simulink model "model"  (R2014a)
(part 7 of 8)

  bus21 : powerlib/Measurements/Load Flow Bus  LConnTagsString=a  ID=bus21  Vbase=50000  Vref=1  Vangle=0  VLF=1  angleLF=0
      settings: AttributesFormatString=|
      | %<ID>
      | %<Vbase>V
      | %<VLF>pu
      | %<angleLF>deg.
      | %<Name>
  bus210 : powerlib/Measurements/Load Flow Bus  LConnTagsString=a  ID=bus210  Vbase=420000  Vref=1  Vangle=0  VLF=1  angleLF=0
      settings: AttributesFormatString=|
      | %<ID>
      | %<Vbase>V
      | %<VLF>pu
      | %<angleLF>deg.
      | %<Name>
  bus211 : powerlib/Measurements/Load Flow Bus  LConnTagsString=a  ID=bus211  Vbase=420000  Vref=1  Vangle=0  VLF=1  angleLF=0
      settings: AttributesFormatString=|
      | %<ID>
      | %<Vbase>V
      | %<VLF>pu
      | %<angleLF>deg.
      | %<Name>
  bus212 : powerlib/Measurements/Load Flow Bus  LConnTagsString=a  ID=bus212  Vbase=420000  Vref=1  Vangle=0  VLF=1  angleLF=0
      settings: AttributesFormatString=|
      | %<ID>
      | %<Vbase>V
      | %<VLF>pu
      | %<angleLF>deg.
      | %<Name>
  bus213 : powerlib/Measurements/Load Flow Bus  LConnTagsString=a  ID=bus213  Vbase=420000  Vref=1  Vangle=0  VLF=1  angleLF=0
      settings: AttributesFormatString=|
      | %<ID>
      | %<Vbase>V
      | %<VLF>pu
      | %<angleLF>deg.
      | %<Name>
  bus214 : powerlib/Measurements/Load Flow Bus  LConnTagsString=a  ID=bus214  Vbase=420000  Vref=1  Vangle=0  VLF=1  angleLF=0
      settings: AttributesFormatString=|
      | %<ID>
      | %<Vbase>V
      | %<VLF>pu
      | %<angleLF>deg.
      | %<Name>
  bus215 : powerlib/Measurements/Load Flow Bus  LConnTagsString=a  ID=bus215  Vbase=420000  Vref=1  Vangle=0  VLF=1  angleLF=0
      settings: AttributesFormatString=|
      | %<ID>
      | %<Vbase>V
      | %<VLF>pu
      | %<angleLF>deg.
      | %<Name>
  bus216 : powerlib/Measurements/Load Flow Bus  LConnTagsString=a  ID=bus216  Vbase=420000  Vref=1  Vangle=0  VLF=1  angleLF=0
      settings: AttributesFormatString=|
      | %<ID>
      | %<Vbase>V
      | %<VLF>pu
      | %<angleLF>deg.
      | %<Name>
  bus217 : powerlib/Measurements/Load Flow Bus  LConnTagsString=a  ID=bus217  Vbase=420000  Vref=1  Vangle=0  VLF=1  angleLF=0
      settings: AttributesFormatString=|
      | %<ID>
      | %<Vbase>V
      | %<VLF>pu
      | %<angleLF>deg.
      | %<Name>
  bus218 : powerlib/Measurements/Load Flow Bus  LConnTagsString=a  ID=bus218  Vbase=420000  Vref=1  Vangle=0  VLF=1  angleLF=0
      settings: AttributesFormatString=|
      | %<ID>
      | %<Vbase>V
      | %<VLF>pu
      | %<angleLF>deg.
      | %<Name>
  bus219 : powerlib/Measurements/Load Flow Bus  LConnTagsString=a  ID=bus219  Vbase=420000  Vref=1  Vangle=0  VLF=1  angleLF=0
      settings: AttributesFormatString=|
      | %<ID>
      | %<Vbase>V
      | %<VLF>pu
      | %<angleLF>deg.
      | %<Name>
  bus22 : powerlib/Measurements/Load Flow Bus  LConnTagsString=a  ID=bus22  Vbase=50000  Vref=1  Vangle=0  VLF=1  angleLF=0
      settings: AttributesFormatString=|
      | %<ID>
      | %<Vbase>V
      | %<VLF>pu
      | %<angleLF>deg.
      | %<Name>
  bus220 : powerlib/Measurements/Load Flow Bus  LConnTagsString=a  ID=bus220  Vbase=420000  Vref=1  Vangle=0  VLF=1  angleLF=0
      settings: AttributesFormatString=|
      | %<ID>
      | %<Vbase>V
      | %<VLF>pu
      | %<angleLF>deg.
      | %<Name>
  bus221 : powerlib/Measurements/Load Flow Bus  LConnTagsString=a  ID=bus221  Vbase=420000  Vref=1  Vangle=0  VLF=1  angleLF=0
      settings: AttributesFormatString=|
      | %<ID>
      | %<Vbase>V
      | %<VLF>pu
      | %<angleLF>deg.
      | %<Name>
  bus222 : powerlib/Measurements/Load Flow Bus  LConnTagsString=a  ID=bus222  Vbase=420000  Vref=1  Vangle=0  VLF=1  angleLF=0
      settings: AttributesFormatString=|
      | %<ID>
      | %<Vbase>V
      | %<VLF>pu
      | %<angleLF>deg.
      | %<Name>
  bus223 : powerlib/Measurements/Load Flow Bus  LConnTagsString=a  ID=bus223  Vbase=420000  Vref=1  Vangle=0  VLF=1  angleLF=0
      settings: AttributesFormatString=|
      | %<ID>
      | %<Vbase>V
      | %<VLF>pu
      | %<angleLF>deg.
      | %<Name>
  bus224 : powerlib/Measurements/Load Flow Bus  LConnTagsString=a  ID=bus224  Vbase=420000  Vref=1  Vangle=0  VLF=1  angleLF=0
      settings: AttributesFormatString=|
      | %<ID>
      | %<Vbase>V
      | %<VLF>pu
      | %<angleLF>deg.
      | %<Name>
  bus225 : powerlib/Measurements/Load Flow Bus  LConnTagsString=a  ID=bus225  Vbase=420000  Vref=1  Vangle=0  VLF=1  angleLF=0
      settings: AttributesFormatString=|
      | %<ID>
      | %<Vbase>V
      | %<VLF>pu
      | %<angleLF>deg.
      | %<Name>
  bus226 : powerlib/Measurements/Load Flow Bus  LConnTagsString=a  ID=bus226  Vbase=420000  Vref=1  Vangle=0  VLF=1  angleLF=0
      settings: AttributesFormatString=|
      | %<ID>
      | %<Vbase>V
      | %<VLF>pu
      | %<angleLF>deg.
      | %<Name>
  bus227 : powerlib/Measurements/Load Flow Bus  LConnTagsString=a  ID=bus227  Vbase=420000  Vref=1  Vangle=0  VLF=1  angleLF=0
      settings: AttributesFormatString=|
      | %<ID>
      | %<Vbase>V
      | %<VLF>pu
      | %<angleLF>deg.
      | %<Name>
  bus228 : powerlib/Measurements/Load Flow Bus  LConnTagsString=a  ID=bus228  Vbase=50000  Vref=1  Vangle=0  VLF=1  angleLF=0
      settings: AttributesFormatString=|
      | %<ID>
      | %<Vbase>V
      | %<VLF>pu
      | %<angleLF>deg.
      | %<Name>
  bus229 : powerlib/Measurements/Load Flow Bus  LConnTagsString=a  ID=bus229  Vbase=50000  Vref=1  Vangle=0  VLF=1  angleLF=0
      settings: AttributesFormatString=|
      | %<ID>
      | %<Vbase>V
      | %<VLF>pu
      | %<angleLF>deg.
      | %<Name>
  bus23 : powerlib/Measurements/Load Flow Bus  LConnTagsString=a  ID=bus23  Vbase=50000  Vref=1  Vangle=0  VLF=1  angleLF=0
      settings: AttributesFormatString=|
      | %<ID>
      | %<Vbase>V
      | %<VLF>pu
      | %<angleLF>deg.
      | %<Name>
  bus230 : powerlib/Measurements/Load Flow Bus  LConnTagsString=a  ID=bus230  Vbase=50000  Vref=1  Vangle=0  VLF=1  angleLF=0
      settings: AttributesFormatString=|
      | %<ID>
      | %<Vbase>V
      | %<VLF>pu
      | %<angleLF>deg.
      | %<Name>
  bus231 : powerlib/Measurements/Load Flow Bus  LConnTagsString=a  ID=bus231  Vbase=50000  Vref=1  Vangle=0  VLF=1  angleLF=0
      settings: AttributesFormatString=|
      | %<ID>
      | %<Vbase>V
      | %<VLF>pu
      | %<angleLF>deg.
      | %<Name>
  bus232 : powerlib/Measurements/Load Flow Bus  LConnTagsString=a  ID=bus232  Vbase=50000  Vref=1  Vangle=0  VLF=1  angleLF=0
      settings: AttributesFormatString=|
      | %<ID>
      | %<Vbase>V
      | %<VLF>pu
      | %<angleLF>deg.
      | %<Name>
  bus233 : powerlib/Measurements/Load Flow Bus  LConnTagsString=a  ID=bus233  Vbase=50000  Vref=1  Vangle=0  VLF=1  angleLF=0
      settings: AttributesFormatString=|
      | %<ID>
      | %<Vbase>V
      | %<VLF>pu
      | %<angleLF>deg.
      | %<Name>
  bus234 : powerlib/Measurements/Load Flow Bus  LConnTagsString=a  ID=bus234  Vbase=50000  Vref=1  Vangle=0  VLF=1  angleLF=0
      settings: AttributesFormatString=|
      | %<ID>
      | %<Vbase>V
      | %<VLF>pu
      | %<angleLF>deg.
      | %<Name>
  bus235 : powerlib/Measurements/Load Flow Bus  LConnTagsString=a  ID=bus235  Vbase=50000  Vref=1  Vangle=0  VLF=1  angleLF=0
      settings: AttributesFormatString=|
      | %<ID>
      | %<Vbase>V
      | %<VLF>pu
      | %<angleLF>deg.
      | %<Name>
  bus236 : powerlib/Measurements/Load Flow Bus  LConnTagsString=a  ID=bus236  Vbase=50000  Vref=1  Vangle=0  VLF=1  angleLF=0
      settings: AttributesFormatString=|
      | %<ID>
      | %<Vbase>V
      | %<VLF>pu
      | %<angleLF>deg.
      | %<Name>
  bus237 : powerlib/Measurements/Load Flow Bus  LConnTagsString=a  ID=bus237  Vbase=50000  Vref=1  Vangle=0  VLF=1  angleLF=0
      settings: AttributesFormatString=|
      | %<ID>
      | %<Vbase>V
      | %<VLF>pu
      | %<angleLF>deg.
      | %<Name>
  bus238 : powerlib/Measurements/Load Flow Bus  LConnTagsString=a  ID=bus238  Vbase=50000  Vref=1  Vangle=0  VLF=1  angleLF=0
      settings: AttributesFormatString=|
      | %<ID>
      | %<Vbase>V
      | %<VLF>pu
      | %<angleLF>deg.
      | %<Name>
  bus239 : powerlib/Measurements/Load Flow Bus  LConnTagsString=a  ID=bus239  Vbase=50000  Vref=1  Vangle=0  VLF=1  angleLF=0
      settings: AttributesFormatString=|
      | %<ID>
      | %<Vbase>V
      | %<VLF>pu
      | %<angleLF>deg.
      | %<Name>
  bus24 : powerlib/Measurements/Load Flow Bus  LConnTagsString=a  ID=bus24  Vbase=50000  Vref=1  Vangle=0  VLF=1  angleLF=0
      settings: AttributesFormatString=|
      | %<ID>
      | %<Vbase>V
      | %<VLF>pu
      | %<angleLF>deg.
      | %<Name>
  bus240 : powerlib/Measurements/Load Flow Bus  LConnTagsString=a  ID=bus240  Vbase=50000  Vref=1  Vangle=0  VLF=1  angleLF=0
      settings: AttributesFormatString=|
      | %<ID>
      | %<Vbase>V
      | %<VLF>pu
      | %<angleLF>deg.
      | %<Name>
  bus241 : powerlib/Measurements/Load Flow Bus  LConnTagsString=a  ID=bus241  Vbase=50000  Vref=1  Vangle=0  VLF=1  angleLF=0
      settings: AttributesFormatString=|
      | %<ID>
      | %<Vbase>V
      | %<VLF>pu
      | %<angleLF>deg.
      | %<Name>
  bus242 : powerlib/Measurements/Load Flow Bus  LConnTagsString=a  ID=bus242  Vbase=50000  Vref=1  Vangle=0  VLF=1  angleLF=0
      settings: AttributesFormatString=|
      | %<ID>
      | %<Vbase>V
      | %<VLF>pu
      | %<angleLF>deg.
      | %<Name>
  bus243 : powerlib/Measurements/Load Flow Bus  LConnTagsString=a  ID=bus243  Vbase=50000  Vref=1  Vangle=0  VLF=1  angleLF=0
      settings: AttributesFormatString=|
      | %<ID>
      | %<Vbase>V
      | %<VLF>pu
      | %<angleLF>deg.
      | %<Name>
  bus244 : powerlib/Measurements/Load Flow Bus  LConnTagsString=a  ID=bus244  Vbase=50000  Vref=1  Vangle=0  VLF=1  angleLF=0
      settings: AttributesFormatString=|
      | %<ID>
      | %<Vbase>V
      | %<VLF>pu
      | %<angleLF>deg.
      | %<Name>
  bus245 : powerlib/Measurements/Load Flow Bus  LConnTagsString=a  ID=bus245  Vbase=50000  Vref=1  Vangle=0  VLF=1  angleLF=0
      settings: AttributesFormatString=|
      | %<ID>
      | %<Vbase>V
      | %<VLF>pu
      | %<angleLF>deg.
      | %<Name>
  bus246 : powerlib/Measurements/Load Flow Bus  LConnTagsString=a  ID=bus246  Vbase=50000  Vref=1  Vangle=0  VLF=1  angleLF=0
      settings: AttributesFormatString=|
      | %<ID>
      | %<Vbase>V
      | %<VLF>pu
      | %<angleLF>deg.
      | %<Name>
  bus247 : powerlib/Measurements/Load Flow Bus  LConnTagsString=a  ID=bus247  Vbase=50000  Vref=1  Vangle=0  VLF=1  angleLF=0
      settings: AttributesFormatString=|
      | %<ID>
      | %<Vbase>V
      | %<VLF>pu
      | %<angleLF>deg.
      | %<Name>
  bus248 : powerlib/Measurements/Load Flow Bus  LConnTagsString=a  ID=bus248  Vbase=50000  Vref=1  Vangle=0  VLF=1  angleLF=0
      settings: AttributesFormatString=|
      | %<ID>
      | %<Vbase>V
      | %<VLF>pu
      | %<angleLF>deg.
      | %<Name>
  bus249 : powerlib/Measurements/Load Flow Bus  LConnTagsString=a  ID=bus249  Vbase=50000  Vref=1  Vangle=0  VLF=1  angleLF=0
      settings: AttributesFormatString=|
      | %<ID>
      | %<Vbase>V
      | %<VLF>pu
      | %<angleLF>deg.
      | %<Name>
  bus25 : powerlib/Measurements/Load Flow Bus  LConnTagsString=a  ID=bus25  Vbase=50000  Vref=1  Vangle=0  VLF=1  angleLF=0
      settings: AttributesFormatString=|
      | %<ID>
      | %<Vbase>V
      | %<VLF>pu
      | %<angleLF>deg.
      | %<Name>
  bus250 : powerlib/Measurements/Load Flow Bus  LConnTagsString=a  ID=bus250  Vbase=50000  Vref=1  Vangle=0  VLF=1  angleLF=0
      settings: AttributesFormatString=|
      | %<ID>
      | %<Vbase>V
      | %<VLF>pu
      | %<angleLF>deg.
      | %<Name>
  bus251 : powerlib/Measurements/Load Flow Bus  LConnTagsString=a  ID=bus251  Vbase=50000  Vref=1  Vangle=0  VLF=1  angleLF=0
      settings: AttributesFormatString=|
      | %<ID>
      | %<Vbase>V
      | %<VLF>pu
      | %<angleLF>deg.
      | %<Name>
  bus252 : powerlib/Measurements/Load Flow Bus  LConnTagsString=a  ID=bus252  Vbase=50000  Vref=1  Vangle=0  VLF=1  angleLF=0
      settings: AttributesFormatString=|
      | %<ID>
      | %<Vbase>V
      | %<VLF>pu
      | %<angleLF>deg.
      | %<Name>
  bus253 : powerlib/Measurements/Load Flow Bus  LConnTagsString=a  ID=bus253  Vbase=50000  Vref=1  Vangle=0  VLF=1  angleLF=0
      settings: AttributesFormatString=|
      | %<ID>
      | %<Vbase>V
      | %<VLF>pu
      | %<angleLF>deg.
      | %<Name>
  bus254 : powerlib/Measurements/Load Flow Bus  LConnTagsString=a  ID=bus254  Vbase=50000  Vref=1  Vangle=0  VLF=1  angleLF=0
      settings: AttributesFormatString=|
      | %<ID>
      | %<Vbase>V
      | %<VLF>pu
      | %<angleLF>deg.
      | %<Name>
  bus255 : powerlib/Measurements/Load Flow Bus  LConnTagsString=a  ID=bus255  Vbase=50000  Vref=1  Vangle=0  VLF=1  angleLF=0
      settings: AttributesFormatString=|
      | %<ID>
      | %<Vbase>V
      | %<VLF>pu
      | %<angleLF>deg.
      | %<Name>
  bus256 : powerlib/Measurements/Load Flow Bus  LConnTagsString=a  ID=bus256  Vbase=66000  Vref=1  Vangle=0  VLF=1  angleLF=0
      settings: AttributesFormatString=|
      | %<ID>
      | %<Vbase>V
      | %<VLF>pu
      | %<angleLF>deg.
      | %<Name>
  bus257 : powerlib/Measurements/Load Flow Bus  LConnTagsString=a  ID=bus257  Vbase=66000  Vref=1  Vangle=0  VLF=1  angleLF=0
      settings: AttributesFormatString=|
      | %<ID>
      | %<Vbase>V
      | %<VLF>pu
      | %<angleLF>deg.
      | %<Name>
  bus258 : powerlib/Measurements/Load Flow Bus  LConnTagsString=a  ID=bus258  Vbase=66000  Vref=1  Vangle=0  VLF=1  angleLF=0
      settings: AttributesFormatString=|
      | %<ID>
      | %<Vbase>V
      | %<VLF>pu
      | %<angleLF>deg.
      | %<Name>
  bus259 : powerlib/Measurements/Load Flow Bus  LConnTagsString=a  ID=bus259  Vbase=66000  Vref=1  Vangle=0  VLF=1  angleLF=0
      settings: AttributesFormatString=|
      | %<ID>
      | %<Vbase>V
      | %<VLF>pu
      | %<angleLF>deg.
      | %<Name>
  bus26 : powerlib/Measurements/Load Flow Bus  LConnTagsString=a  ID=bus26  Vbase=50000  Vref=1  Vangle=0  VLF=1  angleLF=0
      settings: AttributesFormatString=|
      | %<ID>
      | %<Vbase>V
      | %<VLF>pu
      | %<angleLF>deg.
      | %<Name>
  bus260 : powerlib/Measurements/Load Flow Bus  LConnTagsString=a  ID=bus260  Vbase=66000  Vref=1  Vangle=0  VLF=1  angleLF=0
      settings: AttributesFormatString=|
      | %<ID>
      | %<Vbase>V
      | %<VLF>pu
      | %<angleLF>deg.
      | %<Name>
  bus261 : powerlib/Measurements/Load Flow Bus  LConnTagsString=a  ID=bus261  Vbase=66000  Vref=1  Vangle=0  VLF=1  angleLF=0
      settings: AttributesFormatString=|
      | %<ID>
      | %<Vbase>V
      | %<VLF>pu
      | %<angleLF>deg.
      | %<Name>
  bus262 : powerlib/Measurements/Load Flow Bus  LConnTagsString=a  ID=bus262  Vbase=66000  Vref=1  Vangle=0  VLF=1  angleLF=0
      settings: AttributesFormatString=|
      | %<ID>
      | %<Vbase>V
      | %<VLF>pu
      | %<angleLF>deg.
      | %<Name>
  bus263 : powerlib/Measurements/Load Flow Bus  LConnTagsString=a  ID=bus263  Vbase=66000  Vref=1  Vangle=0  VLF=1  angleLF=0
      settings: AttributesFormatString=|
      | %<ID>
      | %<Vbase>V
      | %<VLF>pu
      | %<angleLF>deg.
      | %<Name>
  bus264 : powerlib/Measurements/Load Flow Bus  LConnTagsString=a  ID=bus264  Vbase=66000  Vref=1  Vangle=0  VLF=1  angleLF=0
      settings: AttributesFormatString=|
      | %<ID>
      | %<Vbase>V
      | %<VLF>pu
      | %<angleLF>deg.
      | %<Name>
  bus265 : powerlib/Measurements/Load Flow Bus  LConnTagsString=a  ID=bus265  Vbase=66000  Vref=1  Vangle=0  VLF=1  angleLF=0
      settings: AttributesFormatString=|
      | %<ID>
      | %<Vbase>V
      | %<VLF>pu
      | %<angleLF>deg.
      | %<Name>
  bus266 : powerlib/Measurements/Load Flow Bus  LConnTagsString=a  ID=bus266  Vbase=66000  Vref=1  Vangle=0  VLF=1  angleLF=0
      settings: AttributesFormatString=|
      | %<ID>
      | %<Vbase>V
      | %<VLF>pu
      | %<angleLF>deg.
      | %<Name>
  bus267 : powerlib/Measurements/Load Flow Bus  LConnTagsString=a  ID=bus267  Vbase=66000  Vref=1  Vangle=0  VLF=1  angleLF=0
      settings: AttributesFormatString=|
      | %<ID>
      | %<Vbase>V
      | %<VLF>pu
      | %<angleLF>deg.
      | %<Name>
  bus268 : powerlib/Measurements/Load Flow Bus  LConnTagsString=a  ID=bus268  Vbase=66000  Vref=1  Vangle=0  VLF=1  angleLF=0
      settings: AttributesFormatString=|
      | %<ID>
      | %<Vbase>V
      | %<VLF>pu
      | %<angleLF>deg.
      | %<Name>
  bus269 : powerlib/Measurements/Load Flow Bus  LConnTagsString=a  ID=bus269  Vbase=132000  Vref=1  Vangle=0  VLF=1  angleLF=0
      settings: AttributesFormatString=|
      | %<ID>
      | %<Vbase>V
      | %<VLF>pu
      | %<angleLF>deg.
      | %<Name>
  bus27 : powerlib/Measurements/Load Flow Bus  LConnTagsString=a  ID=bus27  Vbase=50000  Vref=1  Vangle=0  VLF=1  angleLF=0
      settings: AttributesFormatString=|
      | %<ID>
      | %<Vbase>V
      | %<VLF>pu
      | %<angleLF>deg.
      | %<Name>
  bus270 : powerlib/Measurements/Load Flow Bus  LConnTagsString=a  ID=bus270  Vbase=132000  Vref=1  Vangle=0  VLF=1  angleLF=0
      settings: AttributesFormatString=|
      | %<ID>
      | %<Vbase>V
      | %<VLF>pu
      | %<angleLF>deg.
      | %<Name>
  bus271 : powerlib/Measurements/Load Flow Bus  LConnTagsString=a  ID=bus271  Vbase=132000  Vref=1  Vangle=0  VLF=1  angleLF=0
      settings: AttributesFormatString=|
      | %<ID>
      | %<Vbase>V
      | %<VLF>pu
      | %<angleLF>deg.
      | %<Name>
  bus272 : powerlib/Measurements/Load Flow Bus  LConnTagsString=a  ID=bus272  Vbase=132000  Vref=1  Vangle=0  VLF=1  angleLF=0
      settings: AttributesFormatString=|
      | %<ID>
      | %<Vbase>V
      | %<VLF>pu
      | %<angleLF>deg.
      | %<Name>
  bus273 : powerlib/Measurements/Load Flow Bus  LConnTagsString=a  ID=bus273  Vbase=132000  Vref=1  Vangle=0  VLF=1  angleLF=0
      settings: AttributesFormatString=|
      | %<ID>
      | %<Vbase>V
      | %<VLF>pu
      | %<angleLF>deg.
      | %<Name>
  bus274 : powerlib/Measurements/Load Flow Bus  LConnTagsString=a  ID=bus274  Vbase=132000  Vref=1  Vangle=0  VLF=1  angleLF=0
      settings: AttributesFormatString=|
      | %<ID>
      | %<Vbase>V
      | %<VLF>pu
      | %<angleLF>deg.
      | %<Name>
  bus275 : powerlib/Measurements/Load Flow Bus  LConnTagsString=a  ID=bus275  Vbase=132000  Vref=1  Vangle=0  VLF=1  angleLF=0
      settings: AttributesFormatString=|
      | %<ID>
      | %<Vbase>V
      | %<VLF>pu
      | %<angleLF>deg.
      | %<Name>
  bus276 : powerlib/Measurements/Load Flow Bus  LConnTagsString=a  ID=bus276  Vbase=132000  Vref=1  Vangle=0  VLF=1  angleLF=0
      settings: AttributesFormatString=|
      | %<ID>
      | %<Vbase>V
      | %<VLF>pu
      | %<angleLF>deg.
      | %<Name>
  bus277 : powerlib/Measurements/Load Flow Bus  LConnTagsString=a  ID=bus277  Vbase=132000  Vref=1  Vangle=0  VLF=1  angleLF=0
      settings: AttributesFormatString=|
      | %<ID>
      | %<Vbase>V
      | %<VLF>pu
      | %<angleLF>deg.
      | %<Name>
  bus278 : powerlib/Measurements/Load Flow Bus  LConnTagsString=a  ID=bus278  Vbase=132000  Vref=1  Vangle=0  VLF=1  angleLF=0
      settings: AttributesFormatString=|
      | %<ID>
      | %<Vbase>V
      | %<VLF>pu
      | %<angleLF>deg.
      | %<Name>
  bus279 : powerlib/Measurements/Load Flow Bus  LConnTagsString=a  ID=bus279  Vbase=132000  Vref=1  Vangle=0  VLF=1  angleLF=0
      settings: AttributesFormatString=|
      | %<ID>
      | %<Vbase>V
      | %<VLF>pu
      | %<angleLF>deg.
      | %<Name>
  bus28 : powerlib/Measurements/Load Flow Bus  LConnTagsString=a  ID=bus28  Vbase=50000  Vref=1  Vangle=0  VLF=1  angleLF=0
      settings: AttributesFormatString=|
      | %<ID>
      | %<Vbase>V
      | %<VLF>pu
      | %<angleLF>deg.
      | %<Name>
  bus280 : powerlib/Measurements/Load Flow Bus  LConnTagsString=a  ID=bus280  Vbase=132000  Vref=1  Vangle=0  VLF=1  angleLF=0
      settings: AttributesFormatString=|
      | %<ID>
      | %<Vbase>V
      | %<VLF>pu
      | %<angleLF>deg.
      | %<Name>
  bus281 : powerlib/Measurements/Load Flow Bus  LConnTagsString=a  ID=bus281  Vbase=132000  Vref=1  Vangle=0  VLF=1  angleLF=0
      settings: AttributesFormatString=|
      | %<ID>
      | %<Vbase>V
      | %<VLF>pu
      | %<angleLF>deg.
      | %<Name>
  bus282 : powerlib/Measurements/Load Flow Bus  LConnTagsString=a  ID=bus282  Vbase=132000  Vref=1  Vangle=0  VLF=1  angleLF=0
      settings: AttributesFormatString=|
      | %<ID>
      | %<Vbase>V
      | %<VLF>pu
      | %<angleLF>deg.
      | %<Name>
  bus283 : powerlib/Measurements/Load Flow Bus  LConnTagsString=a  ID=bus283  Vbase=132000  Vref=1  Vangle=0  VLF=1  angleLF=0
      settings: AttributesFormatString=|
      | %<ID>
      | %<Vbase>V
      | %<VLF>pu
      | %<angleLF>deg.
      | %<Name>
  bus284 : powerlib/Measurements/Load Flow Bus  LConnTagsString=a  ID=bus284  Vbase=132000  Vref=1  Vangle=0  VLF=1  angleLF=0
      settings: AttributesFormatString=|
      | %<ID>
      | %<Vbase>V
      | %<VLF>pu
      | %<angleLF>deg.
      | %<Name>
  bus285 : powerlib/Measurements/Load Flow Bus  LConnTagsString=a  ID=bus285  Vbase=132000  Vref=1  Vangle=0  VLF=1  angleLF=0
      settings: AttributesFormatString=|
      | %<ID>
      | %<Vbase>V
      | %<VLF>pu
      | %<angleLF>deg.
      | %<Name>
  bus286 : powerlib/Measurements/Load Flow Bus  LConnTagsString=a  ID=bus286  Vbase=132000  Vref=1  Vangle=0  VLF=1  angleLF=0
      settings: AttributesFormatString=|
      | %<ID>
      | %<Vbase>V
      | %<VLF>pu
      | %<angleLF>deg.
      | %<Name>
  bus287 : powerlib/Measurements/Load Flow Bus  LConnTagsString=a  ID=bus287  Vbase=132000  Vref=1  Vangle=0  VLF=1  angleLF=0
      settings: AttributesFormatString=|
      | %<ID>
      | %<Vbase>V
      | %<VLF>pu
      | %<angleLF>deg.
      | %<Name>
  bus288 : powerlib/Measurements/Load Flow Bus  LConnTagsString=a  ID=bus288  Vbase=132000  Vref=1  Vangle=0  VLF=1  angleLF=0
      settings: AttributesFormatString=|
      | %<ID>
      | %<Vbase>V
      | %<VLF>pu
      | %<angleLF>deg.
      | %<Name>
  bus289 : powerlib/Measurements/Load Flow Bus  LConnTagsString=a  ID=bus289  Vbase=132000  Vref=1  Vangle=0  VLF=1  angleLF=0
      settings: AttributesFormatString=|
      | %<ID>
      | %<Vbase>V
      | %<VLF>pu
      | %<angleLF>deg.
      | %<Name>
  bus29 : powerlib/Measurements/Load Flow Bus  LConnTagsString=a  ID=bus29  Vbase=50000  Vref=1  Vangle=0  VLF=1  angleLF=0
      settings: AttributesFormatString=|
      | %<ID>
      | %<Vbase>V
      | %<VLF>pu
      | %<angleLF>deg.
      | %<Name>
  bus290 : powerlib/Measurements/Load Flow Bus  LConnTagsString=a  ID=bus290  Vbase=132000  Vref=1  Vangle=0  VLF=1  angleLF=0
      settings: AttributesFormatString=|
      | %<ID>
      | %<Vbase>V
      | %<VLF>pu
      | %<angleLF>deg.
      | %<Name>
  bus291 : powerlib/Measurements/Load Flow Bus  LConnTagsString=a  ID=bus291  Vbase=132000  Vref=1  Vangle=0  VLF=1  angleLF=0
      settings: AttributesFormatString=|
      | %<ID>
      | %<Vbase>V
      | %<VLF>pu
      | %<angleLF>deg.
      | %<Name>
  bus292 : powerlib/Measurements/Load Flow Bus  LConnTagsString=a  ID=bus292  Vbase=132000  Vref=1  Vangle=0  VLF=1  angleLF=0
      settings: AttributesFormatString=|
      | %<ID>
      | %<Vbase>V
      | %<VLF>pu
      | %<angleLF>deg.
      | %<Name>
  bus293 : powerlib/Measurements/Load Flow Bus  LConnTagsString=a  ID=bus293  Vbase=132000  Vref=1  Vangle=0  VLF=1  angleLF=0
      settings: AttributesFormatString=|
      | %<ID>
      | %<Vbase>V
      | %<VLF>pu
      | %<angleLF>deg.
      | %<Name>
  bus294 : powerlib/Measurements/Load Flow Bus  LConnTagsString=a  ID=bus294  Vbase=132000  Vref=1  Vangle=0  VLF=1  angleLF=0
      settings: AttributesFormatString=|
      | %<ID>
      | %<Vbase>V
      | %<VLF>pu
      | %<angleLF>deg.
      | %<Name>
  bus295 : powerlib/Measurements/Load Flow Bus  LConnTagsString=a  ID=bus295  Vbase=132000  Vref=1  Vangle=0  VLF=1  angleLF=0
      settings: AttributesFormatString=|
      | %<ID>
      | %<Vbase>V
      | %<VLF>pu
      | %<angleLF>deg.
      | %<Name>
  bus296 : powerlib/Measurements/Load Flow Bus  LConnTagsString=a  ID=bus296  Vbase=132000  Vref=1  Vangle=0  VLF=1  angleLF=0
      settings: AttributesFormatString=|
      | %<ID>
      | %<Vbase>V
      | %<VLF>pu
      | %<angleLF>deg.
      | %<Name>
  bus297 : powerlib/Measurements/Load Flow Bus  LConnTagsString=a  ID=bus297  Vbase=132000  Vref=1  Vangle=0  VLF=1  angleLF=0
      settings: AttributesFormatString=|
      | %<ID>
      | %<Vbase>V
      | %<VLF>pu
      | %<angleLF>deg.
      | %<Name>
  bus298 : powerlib/Measurements/Load Flow Bus  LConnTagsString=a  ID=bus298  Vbase=132000  Vref=1  Vangle=0  VLF=1  angleLF=0
      settings: AttributesFormatString=|
      | %<ID>
      | %<Vbase>V
      | %<VLF>pu
      | %<angleLF>deg.
      | %<Name>
  bus299 : powerlib/Measurements/Load Flow Bus  LConnTagsString=a  ID=bus299  Vbase=132000  Vref=1  Vangle=0  VLF=1  angleLF=0
      settings: AttributesFormatString=|
      | %<ID>
      | %<Vbase>V
      | %<VLF>pu
      | %<angleLF>deg.
      | %<Name>
  bus3 : powerlib/Measurements/Load Flow Bus  LConnTagsString=a  ID=bus3  Vbase=50000  Vref=1  Vangle=0  VLF=1  angleLF=0
      settings: AttributesFormatString=|
      | %<ID>
      | %<Vbase>V
      | %<VLF>pu
      | %<angleLF>deg.
      | %<Name>
  bus30 : powerlib/Measurements/Load Flow Bus  LConnTagsString=a  ID=bus30  Vbase=50000  Vref=1  Vangle=0  VLF=1  angleLF=0
      settings: AttributesFormatString=|
      | %<ID>
      | %<Vbase>V
      | %<VLF>pu
      | %<angleLF>deg.
      | %<Name>
  bus300 : powerlib/Measurements/Load Flow Bus  LConnTagsString=a  ID=bus300  Vbase=132000  Vref=1  Vangle=0  VLF=1  angleLF=0
      settings: AttributesFormatString=|
      | %<ID>
      | %<Vbase>V
      | %<VLF>pu
      | %<angleLF>deg.
      | %<Name>
  bus301 : powerlib/Measurements/Load Flow Bus  LConnTagsString=a  ID=bus301  Vbase=132000  Vref=1  Vangle=0  VLF=1  angleLF=0
      settings: AttributesFormatString=|
      | %<ID>
      | %<Vbase>V
      | %<VLF>pu
      | %<angleLF>deg.
      | %<Name>
  bus302 : powerlib/Measurements/Load Flow Bus  LConnTagsString=a  ID=bus302  Vbase=132000  Vref=1  Vangle=0  VLF=1  angleLF=0
      settings: AttributesFormatString=|
      | %<ID>
      | %<Vbase>V
      | %<VLF>pu
      | %<angleLF>deg.
      | %<Name>
  bus303 : powerlib/Measurements/Load Flow Bus  LConnTagsString=a  ID=bus303  Vbase=132000  Vref=1  Vangle=0  VLF=1  angleLF=0
      settings: AttributesFormatString=|
      | %<ID>
      | %<Vbase>V
      | %<VLF>pu
      | %<angleLF>deg.
      | %<Name>
  bus304 : powerlib/Measurements/Load Flow Bus  LConnTagsString=a  ID=bus304  Vbase=132000  Vref=1  Vangle=0  VLF=1  angleLF=0
      settings: AttributesFormatString=|
      | %<ID>
      | %<Vbase>V
      | %<VLF>pu
      | %<angleLF>deg.
      | %<Name>
  bus305 : powerlib/Measurements/Load Flow Bus  LConnTagsString=a  ID=bus305  Vbase=132000  Vref=1  Vangle=0  VLF=1  angleLF=0
      settings: AttributesFormatString=|
      | %<ID>
      | %<Vbase>V
      | %<VLF>pu
      | %<angleLF>deg.
      | %<Name>
  bus306 : powerlib/Measurements/Load Flow Bus  LConnTagsString=a  ID=bus306  Vbase=132000  Vref=1  Vangle=0  VLF=1  angleLF=0
      settings: AttributesFormatString=|
      | %<ID>
      | %<Vbase>V
      | %<VLF>pu
      | %<angleLF>deg.
      | %<Name>
  bus307 : powerlib/Measurements/Load Flow Bus  LConnTagsString=a  ID=bus307  Vbase=132000  Vref=1  Vangle=0  VLF=1  angleLF=0
      settings: AttributesFormatString=|
      | %<ID>
      | %<Vbase>V
      | %<VLF>pu
      | %<angleLF>deg.
      | %<Name>
  bus308 : powerlib/Measurements/Load Flow Bus  LConnTagsString=a  ID=bus308  Vbase=132000  Vref=1  Vangle=0  VLF=1  angleLF=0
      settings: AttributesFormatString=|
      | %<ID>
      | %<Vbase>V
      | %<VLF>pu
      | %<angleLF>deg.
      | %<Name>
  bus309 : powerlib/Measurements/Load Flow Bus  LConnTagsString=a  ID=bus309  Vbase=132000  Vref=1  Vangle=0  VLF=1  angleLF=0
      settings: AttributesFormatString=|
      | %<ID>
      | %<Vbase>V
      | %<VLF>pu
      | %<angleLF>deg.
      | %<Name>
  bus31 : powerlib/Measurements/Load Flow Bus  LConnTagsString=a  ID=bus31  Vbase=50000  Vref=1  Vangle=0  VLF=1  angleLF=0
      settings: AttributesFormatString=|
      | %<ID>
      | %<Vbase>V
      | %<VLF>pu
      | %<angleLF>deg.
      | %<Name>
  bus310 : powerlib/Measurements/Load Flow Bus  LConnTagsString=a  ID=bus310  Vbase=132000  Vref=1  Vangle=0  VLF=1  angleLF=0
      settings: AttributesFormatString=|
      | %<ID>
      | %<Vbase>V
      | %<VLF>pu
      | %<angleLF>deg.
      | %<Name>
  bus311 : powerlib/Measurements/Load Flow Bus  LConnTagsString=a  ID=bus311  Vbase=132000  Vref=1  Vangle=0  VLF=1  angleLF=0
      settings: AttributesFormatString=|
      | %<ID>
      | %<Vbase>V
      | %<VLF>pu
      | %<angleLF>deg.
      | %<Name>
  bus312 : powerlib/Measurements/Load Flow Bus  LConnTagsString=a  ID=bus312  Vbase=132000  Vref=1  Vangle=0  VLF=1  angleLF=0
      settings: AttributesFormatString=|
      | %<ID>
      | %<Vbase>V
      | %<VLF>pu
      | %<angleLF>deg.
      | %<Name>
  bus313 : powerlib/Measurements/Load Flow Bus  LConnTagsString=a  ID=bus313  Vbase=132000  Vref=1  Vangle=0  VLF=1  angleLF=0
      settings: AttributesFormatString=|
      | %<ID>
      | %<Vbase>V
      | %<VLF>pu
      | %<angleLF>deg.
      | %<Name>
  bus314 : powerlib/Measurements/Load Flow Bus  LConnTagsString=a  ID=bus314  Vbase=132000  Vref=1  Vangle=0  VLF=1  angleLF=0
      settings: AttributesFormatString=|
      | %<ID>
      | %<Vbase>V
      | %<VLF>pu
      | %<angleLF>deg.
      | %<Name>
  bus315 : powerlib/Measurements/Load Flow Bus  LConnTagsString=a  ID=bus315  Vbase=132000  Vref=1  Vangle=0  VLF=1  angleLF=0
      settings: AttributesFormatString=|
      | %<ID>
      | %<Vbase>V
      | %<VLF>pu
      | %<angleLF>deg.
      | %<Name>
  bus316 : powerlib/Measurements/Load Flow Bus  LConnTagsString=a  ID=bus316  Vbase=132000  Vref=1  Vangle=0  VLF=1  angleLF=0
      settings: AttributesFormatString=|
      | %<ID>
      | %<Vbase>V
      | %<VLF>pu
      | %<angleLF>deg.
      | %<Name>
  bus317 : powerlib/Measurements/Load Flow Bus  LConnTagsString=a  ID=bus317  Vbase=132000  Vref=1  Vangle=0  VLF=1  angleLF=0
      settings: AttributesFormatString=|
      | %<ID>
      | %<Vbase>V
      | %<VLF>pu
      | %<angleLF>deg.
      | %<Name>
  bus318 : powerlib/Measurements/Load Flow Bus  LConnTagsString=a  ID=bus318  Vbase=132000  Vref=1  Vangle=0  VLF=1  angleLF=0
      settings: AttributesFormatString=|
      | %<ID>
      | %<Vbase>V
      | %<VLF>pu
      | %<angleLF>deg.
      | %<Name>
  bus319 : powerlib/Measurements/Load Flow Bus  LConnTagsString=a  ID=bus319  Vbase=132000  Vref=1  Vangle=0  VLF=1  angleLF=0
      settings: AttributesFormatString=|
      | %<ID>
      | %<Vbase>V
      | %<VLF>pu
      | %<angleLF>deg.
      | %<Name>
  bus32 : powerlib/Measurements/Load Flow Bus  LConnTagsString=a  ID=bus32  Vbase=50000  Vref=1  Vangle=0  VLF=1  angleLF=0
      settings: AttributesFormatString=|
      | %<ID>
      | %<Vbase>V
      | %<VLF>pu
      | %<angleLF>deg.
      | %<Name>
  bus320 : powerlib/Measurements/Load Flow Bus  LConnTagsString=a  ID=bus320  Vbase=132000  Vref=1  Vangle=0  VLF=1  angleLF=0
      settings: AttributesFormatString=|
      | %<ID>
      | %<Vbase>V
      | %<VLF>pu
      | %<angleLF>deg.
      | %<Name>
  bus321 : powerlib/Measurements/Load Flow Bus  LConnTagsString=a  ID=bus321  Vbase=132000  Vref=1  Vangle=0  VLF=1  angleLF=0
      settings: AttributesFormatString=|
      | %<ID>
      | %<Vbase>V
      | %<VLF>pu
      | %<angleLF>deg.
      | %<Name>
  bus322 : powerlib/Measurements/Load Flow Bus  LConnTagsString=a  ID=bus322  Vbase=132000  Vref=1  Vangle=0  VLF=1  angleLF=0
      settings: AttributesFormatString=|
      | %<ID>
      | %<Vbase>V
      | %<VLF>pu
      | %<angleLF>deg.
      | %<Name>
  bus323 : powerlib/Measurements/Load Flow Bus  LConnTagsString=a  ID=bus323  Vbase=132000  Vref=1  Vangle=0  VLF=1  angleLF=0
      settings: AttributesFormatString=|
      | %<ID>
      | %<Vbase>V
      | %<VLF>pu
      | %<angleLF>deg.
      | %<Name>
  bus324 : powerlib/Measurements/Load Flow Bus  LConnTagsString=a  ID=bus324  Vbase=132000  Vref=1  Vangle=0  VLF=1  angleLF=0
      settings: AttributesFormatString=|
      | %<ID>
      | %<Vbase>V
      | %<VLF>pu
      | %<angleLF>deg.
      | %<Name>
  bus325 : powerlib/Measurements/Load Flow Bus  LConnTagsString=a  ID=bus325  Vbase=132000  Vref=1  Vangle=0  VLF=1  angleLF=0
      settings: AttributesFormatString=|
      | %<ID>
      | %<Vbase>V
      | %<VLF>pu
      | %<angleLF>deg.
      | %<Name>
  bus326 : powerlib/Measurements/Load Flow Bus  LConnTagsString=a  ID=bus326  Vbase=132000  Vref=1  Vangle=0  VLF=1  angleLF=0
      settings: AttributesFormatString=|
      | %<ID>
      | %<Vbase>V
      | %<VLF>pu
      | %<angleLF>deg.
      | %<Name>
  bus327 : powerlib/Measurements/Load Flow Bus  LConnTagsString=a  ID=bus327  Vbase=132000  Vref=1  Vangle=0  VLF=1  angleLF=0
      settings: AttributesFormatString=|
      | %<ID>
      | %<Vbase>V
      | %<VLF>pu
      | %<angleLF>deg.
      | %<Name>
  bus328 : powerlib/Measurements/Load Flow Bus  LConnTagsString=a  ID=bus328  Vbase=132000  Vref=1  Vangle=0  VLF=1  angleLF=0
      settings: AttributesFormatString=|
      | %<ID>
      | %<Vbase>V
      | %<VLF>pu
      | %<angleLF>deg.
      | %<Name>
  bus329 : powerlib/Measurements/Load Flow Bus  LConnTagsString=a  ID=bus329  Vbase=132000  Vref=1  Vangle=0  VLF=1  angleLF=0
      settings: AttributesFormatString=|
      | %<ID>
      | %<Vbase>V
      | %<VLF>pu
      | %<angleLF>deg.
      | %<Name>
  bus33 : powerlib/Measurements/Load Flow Bus  LConnTagsString=a  ID=bus33  Vbase=50000  Vref=1  Vangle=0  VLF=1  angleLF=0
      settings: AttributesFormatString=|
      | %<ID>
      | %<Vbase>V
      | %<VLF>pu
      | %<angleLF>deg.
      | %<Name>
  bus330 : powerlib/Measurements/Load Flow Bus  LConnTagsString=a  ID=bus330  Vbase=132000  Vref=1  Vangle=0  VLF=1  angleLF=0
      settings: AttributesFormatString=|
      | %<ID>
      | %<Vbase>V
      | %<VLF>pu
      | %<angleLF>deg.
      | %<Name>
  bus331 : powerlib/Measurements/Load Flow Bus  LConnTagsString=a  ID=bus331  Vbase=132000  Vref=1  Vangle=0  VLF=1  angleLF=0
      settings: AttributesFormatString=|
      | %<ID>
      | %<Vbase>V
      | %<VLF>pu
      | %<angleLF>deg.
      | %<Name>
  bus332 : powerlib/Measurements/Load Flow Bus  LConnTagsString=a  ID=bus332  Vbase=132000  Vref=1  Vangle=0  VLF=1  angleLF=0
      settings: AttributesFormatString=|
      | %<ID>
      | %<Vbase>V
      | %<VLF>pu
      | %<angleLF>deg.
      | %<Name>
  bus333 : powerlib/Measurements/Load Flow Bus  LConnTagsString=a  ID=bus333  Vbase=132000  Vref=1  Vangle=0  VLF=1  angleLF=0
      settings: AttributesFormatString=|
      | %<ID>
      | %<Vbase>V
      | %<VLF>pu
      | %<angleLF>deg.
      | %<Name>
  bus334 : powerlib/Measurements/Load Flow Bus  LConnTagsString=a  ID=bus334  Vbase=132000  Vref=1  Vangle=0  VLF=1  angleLF=0
      settings: AttributesFormatString=|
      | %<ID>
      | %<Vbase>V
      | %<VLF>pu
      | %<angleLF>deg.
      | %<Name>
  bus335 : powerlib/Measurements/Load Flow Bus  LConnTagsString=a  ID=bus335  Vbase=132000  Vref=1  Vangle=0  VLF=1  angleLF=0
      settings: AttributesFormatString=|
      | %<ID>
      | %<Vbase>V
      | %<VLF>pu
      | %<angleLF>deg.
      | %<Name>
  bus336 : powerlib/Measurements/Load Flow Bus  LConnTagsString=a  ID=bus336  Vbase=300000  Vref=1  Vangle=0  VLF=1  angleLF=0
      settings: AttributesFormatString=|
      | %<ID>
      | %<Vbase>V
      | %<VLF>pu
      | %<angleLF>deg.
      | %<Name>
  bus337 : powerlib/Measurements/Load Flow Bus  LConnTagsString=a  ID=bus337  Vbase=300000  Vref=1  Vangle=0  VLF=1  angleLF=0
      settings: AttributesFormatString=|
      | %<ID>
      | %<Vbase>V
      | %<VLF>pu
      | %<angleLF>deg.
      | %<Name>
  bus338 : powerlib/Measurements/Load Flow Bus  LConnTagsString=a  ID=bus338  Vbase=300000  Vref=1  Vangle=0  VLF=1  angleLF=0
      settings: AttributesFormatString=|
      | %<ID>
      | %<Vbase>V
      | %<VLF>pu
      | %<angleLF>deg.
      | %<Name>
  bus339 : powerlib/Measurements/Load Flow Bus  LConnTagsString=a  ID=bus339  Vbase=300000  Vref=1  Vangle=0  VLF=1  angleLF=0
      settings: AttributesFormatString=|
      | %<ID>
      | %<Vbase>V
      | %<VLF>pu
      | %<angleLF>deg.
      | %<Name>
  bus34 : powerlib/Measurements/Load Flow Bus  LConnTagsString=a  ID=bus34  Vbase=66000  Vref=1  Vangle=0  VLF=1  angleLF=0
      settings: AttributesFormatString=|
      | %<ID>
      | %<Vbase>V
      | %<VLF>pu
      | %<angleLF>deg.
      | %<Name>
  bus340 : powerlib/Measurements/Load Flow Bus  LConnTagsString=a  ID=bus340  Vbase=300000  Vref=1  Vangle=0  VLF=1  angleLF=0
      settings: AttributesFormatString=|
      | %<ID>
      | %<Vbase>V
      | %<VLF>pu
      | %<angleLF>deg.
      | %<Name>
  bus341 : powerlib/Measurements/Load Flow Bus  LConnTagsString=a  ID=bus341  Vbase=300000  Vref=1  Vangle=0  VLF=1  angleLF=0
      settings: AttributesFormatString=|
      | %<ID>
      | %<Vbase>V
      | %<VLF>pu
      | %<angleLF>deg.
      | %<Name>
  bus342 : powerlib/Measurements/Load Flow Bus  LConnTagsString=a  ID=bus342  Vbase=300000  Vref=1  Vangle=0  VLF=1  angleLF=0
      settings: AttributesFormatString=|
      | %<ID>
      | %<Vbase>V
      | %<VLF>pu
      | %<angleLF>deg.
      | %<Name>
  bus343 : powerlib/Measurements/Load Flow Bus  LConnTagsString=a  ID=bus343  Vbase=300000  Vref=1  Vangle=0  VLF=1  angleLF=0
      settings: AttributesFormatString=|
      | %<ID>
      | %<Vbase>V
      | %<VLF>pu
      | %<angleLF>deg.
      | %<Name>
  bus344 : powerlib/Measurements/Load Flow Bus  LConnTagsString=a  ID=bus344  Vbase=300000  Vref=1  Vangle=0  VLF=1  angleLF=0
      settings: AttributesFormatString=|
      | %<ID>
      | %<Vbase>V
      | %<VLF>pu
      | %<angleLF>deg.
      | %<Name>
  bus345 : powerlib/Measurements/Load Flow Bus  LConnTagsString=a  ID=bus345  Vbase=300000  Vref=1  Vangle=0  VLF=1  angleLF=0
      settings: AttributesFormatString=|
      | %<ID>
      | %<Vbase>V
      | %<VLF>pu
      | %<angleLF>deg.
      | %<Name>
  bus346 : powerlib/Measurements/Load Flow Bus  LConnTagsString=a  ID=bus346  Vbase=300000  Vref=1  Vangle=0  VLF=1  angleLF=0
      settings: AttributesFormatString=|
      | %<ID>
      | %<Vbase>V
      | %<VLF>pu
      | %<angleLF>deg.
      | %<Name>
  bus347 : powerlib/Measurements/Load Flow Bus  LConnTagsString=a  ID=bus347  Vbase=300000  Vref=1  Vangle=0  VLF=1  angleLF=0
      settings: AttributesFormatString=|
      | %<ID>
      | %<Vbase>V
      | %<VLF>pu
      | %<angleLF>deg.
      | %<Name>
  bus348 : powerlib/Measurements/Load Flow Bus  LConnTagsString=a  ID=bus348  Vbase=300000  Vref=1  Vangle=0  VLF=1  angleLF=0
      settings: AttributesFormatString=|
      | %<ID>
      | %<Vbase>V
      | %<VLF>pu
      | %<angleLF>deg.
      | %<Name>
  bus349 : powerlib/Measurements/Load Flow Bus  LConnTagsString=a  ID=bus349  Vbase=300000  Vref=1  Vangle=0  VLF=1  angleLF=0
      settings: AttributesFormatString=|
      | %<ID>
      | %<Vbase>V
      | %<VLF>pu
      | %<angleLF>deg.
      | %<Name>
  bus35 : powerlib/Measurements/Load Flow Bus  LConnTagsString=a  ID=bus35  Vbase=66000  Vref=1  Vangle=0  VLF=1  angleLF=0
      settings: AttributesFormatString=|
      | %<ID>
      | %<Vbase>V
      | %<VLF>pu
      | %<angleLF>deg.
      | %<Name>
  bus350 : powerlib/Measurements/Load Flow Bus  LConnTagsString=a  ID=bus350  Vbase=300000  Vref=1  Vangle=0  VLF=1  angleLF=0
      settings: AttributesFormatString=|
      | %<ID>
      | %<Vbase>V
      | %<VLF>pu
      | %<angleLF>deg.
      | %<Name>
  bus351 : powerlib/Measurements/Load Flow Bus  LConnTagsString=a  ID=bus351  Vbase=300000  Vref=1  Vangle=0  VLF=1  angleLF=0
      settings: AttributesFormatString=|
      | %<ID>
      | %<Vbase>V
      | %<VLF>pu
      | %<angleLF>deg.
      | %<Name>
  bus352 : powerlib/Measurements/Load Flow Bus  LConnTagsString=a  ID=bus352  Vbase=300000  Vref=1  Vangle=0  VLF=1  angleLF=0
      settings: AttributesFormatString=|
      | %<ID>
      | %<Vbase>V
      | %<VLF>pu
      | %<angleLF>deg.
      | %<Name>
  bus353 : powerlib/Measurements/Load Flow Bus  LConnTagsString=a  ID=bus353  Vbase=300000  Vref=1  Vangle=0  VLF=1  angleLF=0
      settings: AttributesFormatString=|
      | %<ID>
      | %<Vbase>V
      | %<VLF>pu
      | %<angleLF>deg.
      | %<Name>
  bus354 : powerlib/Measurements/Load Flow Bus  LConnTagsString=a  ID=bus354  Vbase=300000  Vref=1  Vangle=0  VLF=1  angleLF=0
      settings: AttributesFormatString=|
      | %<ID>
      | %<Vbase>V
      | %<VLF>pu
      | %<angleLF>deg.
      | %<Name>
  bus355 : powerlib/Measurements/Load Flow Bus  LConnTagsString=a  ID=bus355  Vbase=300000  Vref=1  Vangle=0  VLF=1  angleLF=0
      settings: AttributesFormatString=|
      | %<ID>
      | %<Vbase>V
      | %<VLF>pu
      | %<angleLF>deg.
      | %<Name>
  bus356 : powerlib/Measurements/Load Flow Bus  LConnTagsString=a  ID=bus356  Vbase=300000  Vref=1  Vangle=0  VLF=1  angleLF=0
      settings: AttributesFormatString=|
      | %<ID>
      | %<Vbase>V
      | %<VLF>pu
      | %<angleLF>deg.
      | %<Name>
  bus357 : powerlib/Measurements/Load Flow Bus  LConnTagsString=a  ID=bus357  Vbase=300000  Vref=1  Vangle=0  VLF=1  angleLF=0
      settings: AttributesFormatString=|
      | %<ID>
      | %<Vbase>V
      | %<VLF>pu
      | %<angleLF>deg.
      | %<Name>
  bus358 : powerlib/Measurements/Load Flow Bus  LConnTagsString=a  ID=bus358  Vbase=300000  Vref=1  Vangle=0  VLF=1  angleLF=0
      settings: AttributesFormatString=|
      | %<ID>
      | %<Vbase>V
      | %<VLF>pu
      | %<angleLF>deg.
      | %<Name>
  bus359 : powerlib/Measurements/Load Flow Bus  LConnTagsString=a  ID=bus359  Vbase=300000  Vref=1  Vangle=0  VLF=1  angleLF=0
      settings: AttributesFormatString=|
      | %<ID>
      | %<Vbase>V
      | %<VLF>pu
      | %<angleLF>deg.
      | %<Name>
  bus36 : powerlib/Measurements/Load Flow Bus  LConnTagsString=a  ID=bus36  Vbase=66000  Vref=1  Vangle=0  VLF=1  angleLF=0
      settings: AttributesFormatString=|
      | %<ID>
      | %<Vbase>V
      | %<VLF>pu
      | %<angleLF>deg.
      | %<Name>
  bus360 : powerlib/Measurements/Load Flow Bus  LConnTagsString=a  ID=bus360  Vbase=300000  Vref=1  Vangle=0  VLF=1  angleLF=0
      settings: AttributesFormatString=|
      | %<ID>
      | %<Vbase>V
      | %<VLF>pu
      | %<angleLF>deg.
      | %<Name>
  bus361 : powerlib/Measurements/Load Flow Bus  LConnTagsString=a  ID=bus361  Vbase=300000  Vref=1  Vangle=0  VLF=1  angleLF=0
      settings: AttributesFormatString=|
      | %<ID>
      | %<Vbase>V
      | %<VLF>pu
      | %<angleLF>deg.
      | %<Name>
  bus362 : powerlib/Measurements/Load Flow Bus  LConnTagsString=a  ID=bus362  Vbase=300000  Vref=1  Vangle=0  VLF=1  angleLF=0
      settings: AttributesFormatString=|
      | %<ID>
      | %<Vbase>V
      | %<VLF>pu
      | %<angleLF>deg.
      | %<Name>
  bus363 : powerlib/Measurements/Load Flow Bus  LConnTagsString=a  ID=bus363  Vbase=300000  Vref=1  Vangle=0  VLF=1  angleLF=0
      settings: AttributesFormatString=|
      | %<ID>
      | %<Vbase>V
      | %<VLF>pu
      | %<angleLF>deg.
      | %<Name>
  bus364 : powerlib/Measurements/Load Flow Bus  LConnTagsString=a  ID=bus364  Vbase=300000  Vref=1  Vangle=0  VLF=1  angleLF=0
      settings: AttributesFormatString=|
      | %<ID>
      | %<Vbase>V
      | %<VLF>pu
      | %<angleLF>deg.
      | %<Name>
  bus365 : powerlib/Measurements/Load Flow Bus  LConnTagsString=a  ID=bus365  Vbase=300000  Vref=1  Vangle=0  VLF=1  angleLF=0
      settings: AttributesFormatString=|
      | %<ID>
      | %<Vbase>V
      | %<VLF>pu
      | %<angleLF>deg.
      | %<Name>
  bus366 : powerlib/Measurements/Load Flow Bus  LConnTagsString=a  ID=bus366  Vbase=300000  Vref=1  Vangle=0  VLF=1  angleLF=0
      settings: AttributesFormatString=|
      | %<ID>
      | %<Vbase>V
      | %<VLF>pu
      | %<angleLF>deg.
      | %<Name>
  bus367 : powerlib/Measurements/Load Flow Bus  LConnTagsString=a  ID=bus367  Vbase=300000  Vref=1  Vangle=0  VLF=1  angleLF=0
      settings: AttributesFormatString=|
      | %<ID>
      | %<Vbase>V
      | %<VLF>pu
      | %<angleLF>deg.
      | %<Name>
  bus368 : powerlib/Measurements/Load Flow Bus  LConnTagsString=a  ID=bus368  Vbase=300000  Vref=1  Vangle=0  VLF=1  angleLF=0
      settings: AttributesFormatString=|
      | %<ID>
      | %<Vbase>V
      | %<VLF>pu
      | %<angleLF>deg.
      | %<Name>
  bus369 : powerlib/Measurements/Load Flow Bus  LConnTagsString=a  ID=bus369  Vbase=300000  Vref=1  Vangle=0  VLF=1  angleLF=0
      settings: AttributesFormatString=|
      | %<ID>
      | %<Vbase>V
      | %<VLF>pu
      | %<angleLF>deg.
      | %<Name>
  bus37 : powerlib/Measurements/Load Flow Bus  LConnTagsString=a  ID=bus37  Vbase=66000  Vref=1  Vangle=0  VLF=1  angleLF=0
      settings: AttributesFormatString=|
      | %<ID>
      | %<Vbase>V
      | %<VLF>pu
      | %<angleLF>deg.
      | %<Name>
  bus370 : powerlib/Measurements/Load Flow Bus  LConnTagsString=a  ID=bus370  Vbase=300000  Vref=1  Vangle=0  VLF=1  angleLF=0
      settings: AttributesFormatString=|
      | %<ID>
      | %<Vbase>V
      | %<VLF>pu
      | %<angleLF>deg.
      | %<Name>
  bus371 : powerlib/Measurements/Load Flow Bus  LConnTagsString=a  ID=bus371  Vbase=300000  Vref=1  Vangle=0  VLF=1  angleLF=0
      settings: AttributesFormatString=|
      | %<ID>
      | %<Vbase>V
      | %<VLF>pu
      | %<angleLF>deg.
      | %<Name>
  bus372 : powerlib/Measurements/Load Flow Bus  LConnTagsString=a  ID=bus372  Vbase=300000  Vref=1  Vangle=0  VLF=1  angleLF=0
      settings: AttributesFormatString=|
      | %<ID>
      | %<Vbase>V
      | %<VLF>pu
      | %<angleLF>deg.
      | %<Name>
  bus373 : powerlib/Measurements/Load Flow Bus  LConnTagsString=a  ID=bus373  Vbase=300000  Vref=1  Vangle=0  VLF=1  angleLF=0
      settings: AttributesFormatString=|
      | %<ID>
      | %<Vbase>V
      | %<VLF>pu
      | %<angleLF>deg.
      | %<Name>
  bus374 : powerlib/Measurements/Load Flow Bus  LConnTagsString=a  ID=bus374  Vbase=300000  Vref=1  Vangle=0  VLF=1  angleLF=0
      settings: AttributesFormatString=|
      | %<ID>
      | %<Vbase>V
      | %<VLF>pu
      | %<angleLF>deg.
      | %<Name>
  bus375 : powerlib/Measurements/Load Flow Bus  LConnTagsString=a  ID=bus375  Vbase=300000  Vref=1  Vangle=0  VLF=1  angleLF=0
      settings: AttributesFormatString=|
      | %<ID>
      | %<Vbase>V
      | %<VLF>pu
      | %<angleLF>deg.
      | %<Name>
  bus376 : powerlib/Measurements/Load Flow Bus  LConnTagsString=a  ID=bus376  Vbase=300000  Vref=1  Vangle=0  VLF=1  angleLF=0
      settings: AttributesFormatString=|
      | %<ID>
      | %<Vbase>V
      | %<VLF>pu
      | %<angleLF>deg.
      | %<Name>
  bus377 : powerlib/Measurements/Load Flow Bus  LConnTagsString=a  ID=bus377  Vbase=300000  Vref=1  Vangle=0  VLF=1  angleLF=0
      settings: AttributesFormatString=|
      | %<ID>
      | %<Vbase>V
      | %<VLF>pu
      | %<angleLF>deg.
      | %<Name>
  bus378 : powerlib/Measurements/Load Flow Bus  LConnTagsString=a  ID=bus378  Vbase=300000  Vref=1  Vangle=0  VLF=1  angleLF=0
      settings: AttributesFormatString=|
      | %<ID>
      | %<Vbase>V
      | %<VLF>pu
      | %<angleLF>deg.
      | %<Name>
  bus379 : powerlib/Measurements/Load Flow Bus  LConnTagsString=a  ID=bus379  Vbase=420000  Vref=1  Vangle=0  VLF=1  angleLF=0
      settings: AttributesFormatString=|
      | %<ID>
      | %<Vbase>V
      | %<VLF>pu
      | %<angleLF>deg.
      | %<Name>
  bus38 : powerlib/Measurements/Load Flow Bus  LConnTagsString=a  ID=bus38  Vbase=66000  Vref=1  Vangle=0  VLF=1  angleLF=0
      settings: AttributesFormatString=|
      | %<ID>
      | %<Vbase>V
      | %<VLF>pu
      | %<angleLF>deg.
      | %<Name>
  bus380 : powerlib/Measurements/Load Flow Bus  LConnTagsString=a  ID=bus380  Vbase=420000  Vref=1  Vangle=0  VLF=1  angleLF=0
      settings: AttributesFormatString=|
      | %<ID>
      | %<Vbase>V
      | %<VLF>pu
      | %<angleLF>deg.
      | %<Name>
  bus381 : powerlib/Measurements/Load Flow Bus  LConnTagsString=a  ID=bus381  Vbase=420000  Vref=1  Vangle=0  VLF=1  angleLF=0
      settings: AttributesFormatString=|
      | %<ID>
      | %<Vbase>V
      | %<VLF>pu
      | %<angleLF>deg.
      | %<Name>
  bus382 : powerlib/Measurements/Load Flow Bus  LConnTagsString=a  ID=bus382  Vbase=420000  Vref=1  Vangle=0  VLF=1  angleLF=0
      settings: AttributesFormatString=|
      | %<ID>
      | %<Vbase>V
      | %<VLF>pu
      | %<angleLF>deg.
      | %<Name>
  bus383 : powerlib/Measurements/Load Flow Bus  LConnTagsString=a  ID=bus383  Vbase=420000  Vref=1  Vangle=0  VLF=1  angleLF=0
      settings: AttributesFormatString=|
      | %<ID>
      | %<Vbase>V
      | %<VLF>pu
      | %<angleLF>deg.
      | %<Name>
  bus384 : powerlib/Measurements/Load Flow Bus  LConnTagsString=a  ID=bus384  Vbase=420000  Vref=1  Vangle=0  VLF=1  angleLF=0
      settings: AttributesFormatString=|
      | %<ID>
      | %<Vbase>V
      | %<VLF>pu
      | %<angleLF>deg.
      | %<Name>
  bus385 : powerlib/Measurements/Load Flow Bus  LConnTagsString=a  ID=bus385  Vbase=420000  Vref=1  Vangle=0  VLF=1  angleLF=0
      settings: AttributesFormatString=|
      | %<ID>
      | %<Vbase>V
      | %<VLF>pu
      | %<angleLF>deg.
      | %<Name>
  bus386 : powerlib/Measurements/Load Flow Bus  LConnTagsString=a  ID=bus386  Vbase=420000  Vref=1  Vangle=0  VLF=1  angleLF=0
      settings: AttributesFormatString=|
      | %<ID>
      | %<Vbase>V
      | %<VLF>pu
      | %<angleLF>deg.
      | %<Name>
  bus387 : powerlib/Measurements/Load Flow Bus  LConnTagsString=a  ID=bus387  Vbase=420000  Vref=1  Vangle=0  VLF=1  angleLF=0
      settings: AttributesFormatString=|
      | %<ID>
      | %<Vbase>V
      | %<VLF>pu
      | %<angleLF>deg.
      | %<Name>
  bus388 : powerlib/Measurements/Load Flow Bus  LConnTagsString=a  ID=bus388  Vbase=420000  Vref=1  Vangle=0  VLF=1  angleLF=0
      settings: AttributesFormatString=|
      | %<ID>
      | %<Vbase>V
      | %<VLF>pu
      | %<angleLF>deg.
      | %<Name>
  bus389 : powerlib/Measurements/Load Flow Bus  LConnTagsString=a  ID=bus389  Vbase=420000  Vref=1  Vangle=0  VLF=1  angleLF=0
      settings: AttributesFormatString=|
      | %<ID>
      | %<Vbase>V
      | %<VLF>pu
      | %<angleLF>deg.
      | %<Name>
  bus39 : powerlib/Measurements/Load Flow Bus  LConnTagsString=a  ID=bus39  Vbase=66000  Vref=1  Vangle=0  VLF=1  angleLF=0
      settings: AttributesFormatString=|
      | %<ID>
      | %<Vbase>V
      | %<VLF>pu
      | %<angleLF>deg.
      | %<Name>
  bus390 : powerlib/Measurements/Load Flow Bus  LConnTagsString=a  ID=bus390  Vbase=420000  Vref=1  Vangle=0  VLF=1  angleLF=0
      settings: AttributesFormatString=|
      | %<ID>
      | %<Vbase>V
      | %<VLF>pu
      | %<angleLF>deg.
      | %<Name>
  bus391 : powerlib/Measurements/Load Flow Bus  LConnTagsString=a  ID=bus391  Vbase=420000  Vref=1  Vangle=0  VLF=1  angleLF=0
      settings: AttributesFormatString=|
      | %<ID>
      | %<Vbase>V
      | %<VLF>pu
      | %<angleLF>deg.
      | %<Name>
  bus392 : powerlib/Measurements/Load Flow Bus  LConnTagsString=a  ID=bus392  Vbase=420000  Vref=1  Vangle=0  VLF=1  angleLF=0
      settings: AttributesFormatString=|
      | %<ID>
      | %<Vbase>V
      | %<VLF>pu
      | %<angleLF>deg.
      | %<Name>
  bus393 : powerlib/Measurements/Load Flow Bus  LConnTagsString=a  ID=bus393  Vbase=420000  Vref=1  Vangle=0  VLF=1  angleLF=0
      settings: AttributesFormatString=|
      | %<ID>
      | %<Vbase>V
      | %<VLF>pu
      | %<angleLF>deg.
      | %<Name>
  bus4 : powerlib/Measurements/Load Flow Bus  LConnTagsString=a  ID=bus4  Vbase=50000  Vref=1  Vangle=0  VLF=1  angleLF=0
      settings: AttributesFormatString=|
      | %<ID>
      | %<Vbase>V
      | %<VLF>pu
      | %<angleLF>deg.
      | %<Name>
  bus40 : powerlib/Measurements/Load Flow Bus  LConnTagsString=a  ID=bus40  Vbase=66000  Vref=1  Vangle=0  VLF=1  angleLF=0
      settings: AttributesFormatString=|
      | %<ID>
      | %<Vbase>V
      | %<VLF>pu
      | %<angleLF>deg.
      | %<Name>
  bus41 : powerlib/Measurements/Load Flow Bus  LConnTagsString=a  ID=bus41  Vbase=66000  Vref=1  Vangle=0  VLF=1  angleLF=0
      settings: AttributesFormatString=|
      | %<ID>
      | %<Vbase>V
      | %<VLF>pu
      | %<angleLF>deg.
      | %<Name>
  bus42 : powerlib/Measurements/Load Flow Bus  LConnTagsString=a  ID=bus42  Vbase=66000  Vref=1  Vangle=0  VLF=1  angleLF=0
      settings: AttributesFormatString=|
      | %<ID>
      | %<Vbase>V
      | %<VLF>pu
      | %<angleLF>deg.
      | %<Name>
  bus43 : powerlib/Measurements/Load Flow Bus  LConnTagsString=a  ID=bus43  Vbase=66000  Vref=1  Vangle=0  VLF=1  angleLF=0
      settings: AttributesFormatString=|
      | %<ID>
      | %<Vbase>V
      | %<VLF>pu
      | %<angleLF>deg.
      | %<Name>
  bus44 : powerlib/Measurements/Load Flow Bus  LConnTagsString=a  ID=bus44  Vbase=66000  Vref=1  Vangle=0  VLF=1  angleLF=0
      settings: AttributesFormatString=|
      | %<ID>
      | %<Vbase>V
      | %<VLF>pu
      | %<angleLF>deg.
      | %<Name>
  bus45 : powerlib/Measurements/Load Flow Bus  LConnTagsString=a  ID=bus45  Vbase=66000  Vref=1  Vangle=0  VLF=1  angleLF=0
      settings: AttributesFormatString=|
      | %<ID>
      | %<Vbase>V
      | %<VLF>pu
      | %<angleLF>deg.
      | %<Name>
  bus46 : powerlib/Measurements/Load Flow Bus  LConnTagsString=a  ID=bus46  Vbase=66000  Vref=1  Vangle=0  VLF=1  angleLF=0
      settings: AttributesFormatString=|
      | %<ID>
      | %<Vbase>V
      | %<VLF>pu
      | %<angleLF>deg.
      | %<Name>
  bus47 : powerlib/Measurements/Load Flow Bus  LConnTagsString=a  ID=bus47  Vbase=66000  Vref=1  Vangle=0  VLF=1  angleLF=0
      settings: AttributesFormatString=|
      | %<ID>
      | %<Vbase>V
      | %<VLF>pu
      | %<angleLF>deg.
      | %<Name>
  bus48 : powerlib/Measurements/Load Flow Bus  LConnTagsString=a  ID=bus48  Vbase=66000  Vref=1  Vangle=0  VLF=1  angleLF=0
      settings: AttributesFormatString=|
      | %<ID>
      | %<Vbase>V
      | %<VLF>pu
      | %<angleLF>deg.
      | %<Name>
  bus49 : powerlib/Measurements/Load Flow Bus  LConnTagsString=a  ID=bus49  Vbase=66000  Vref=1  Vangle=0  VLF=1  angleLF=0
      settings: AttributesFormatString=|
      | %<ID>
      | %<Vbase>V
      | %<VLF>pu
      | %<angleLF>deg.
      | %<Name>
  bus5 : powerlib/Measurements/Load Flow Bus  LConnTagsString=a  ID=bus5  Vbase=50000  Vref=1  Vangle=0  VLF=1  angleLF=0
      settings: AttributesFormatString=|
      | %<ID>
      | %<Vbase>V
      | %<VLF>pu
      | %<angleLF>deg.
      | %<Name>
  bus50 : powerlib/Measurements/Load Flow Bus  LConnTagsString=a  ID=bus50  Vbase=66000  Vref=1  Vangle=0  VLF=1  angleLF=0
      settings: AttributesFormatString=|
      | %<ID>
      | %<Vbase>V
      | %<VLF>pu
      | %<angleLF>deg.
      | %<Name>
  bus51 : powerlib/Measurements/Load Flow Bus  LConnTagsString=a  ID=bus51  Vbase=132000  Vref=1  Vangle=0  VLF=1  angleLF=0
      settings: AttributesFormatString=|
      | %<ID>
      | %<Vbase>V
      | %<VLF>pu
      | %<angleLF>deg.
      | %<Name>
  bus52 : powerlib/Measurements/Load Flow Bus  LConnTagsString=a  ID=bus52  Vbase=132000  Vref=1  Vangle=0  VLF=1  angleLF=0
      settings: AttributesFormatString=|
      | %<ID>
      | %<Vbase>V
      | %<VLF>pu
      | %<angleLF>deg.
      | %<Name>
  bus53 : powerlib/Measurements/Load Flow Bus  LConnTagsString=a  ID=bus53  Vbase=132000  Vref=1  Vangle=0  VLF=1  angleLF=0
      settings: AttributesFormatString=|
      | %<ID>
      | %<Vbase>V
      | %<VLF>pu
      | %<angleLF>deg.
      | %<Name>
  bus54 : powerlib/Measurements/Load Flow Bus  LConnTagsString=a  ID=bus54  Vbase=132000  Vref=1  Vangle=0  VLF=1  angleLF=0
      settings: AttributesFormatString=|
      | %<ID>
      | %<Vbase>V
      | %<VLF>pu
      | %<angleLF>deg.
      | %<Name>
  bus55 : powerlib/Measurements/Load Flow Bus  LConnTagsString=a  ID=bus55  Vbase=132000  Vref=1  Vangle=0  VLF=1  angleLF=0
      settings: AttributesFormatString=|
      | %<ID>
      | %<Vbase>V
      | %<VLF>pu
      | %<angleLF>deg.
      | %<Name>
  bus56 : powerlib/Measurements/Load Flow Bus  LConnTagsString=a  ID=bus56  Vbase=132000  Vref=1  Vangle=0  VLF=1  angleLF=0
      settings: AttributesFormatString=|
      | %<ID>
      | %<Vbase>V
      | %<VLF>pu
      | %<angleLF>deg.
      | %<Name>
  bus57 : powerlib/Measurements/Load Flow Bus  LConnTagsString=a  ID=bus57  Vbase=132000  Vref=1  Vangle=0  VLF=1  angleLF=0
      settings: AttributesFormatString=|
      | %<ID>
      | %<Vbase>V
      | %<VLF>pu
      | %<angleLF>deg.
      | %<Name>
  bus58 : powerlib/Measurements/Load Flow Bus  LConnTagsString=a  ID=bus58  Vbase=132000  Vref=1  Vangle=0  VLF=1  angleLF=0
      settings: AttributesFormatString=|
      | %<ID>
      | %<Vbase>V
      | %<VLF>pu
      | %<angleLF>deg.
      | %<Name>
  bus59 : powerlib/Measurements/Load Flow Bus  LConnTagsString=a  ID=bus59  Vbase=132000  Vref=1  Vangle=0  VLF=1  angleLF=0
      settings: AttributesFormatString=|
      | %<ID>
      | %<Vbase>V
      | %<VLF>pu
      | %<angleLF>deg.
      | %<Name>
  bus6 : powerlib/Measurements/Load Flow Bus  LConnTagsString=a  ID=bus6  Vbase=50000  Vref=1  Vangle=0  VLF=1  angleLF=0
      settings: AttributesFormatString=|
      | %<ID>
      | %<Vbase>V
      | %<VLF>pu
      | %<angleLF>deg.
      | %<Name>
  bus60 : powerlib/Measurements/Load Flow Bus  LConnTagsString=a  ID=bus60  Vbase=132000  Vref=1  Vangle=0  VLF=1  angleLF=0
      settings: AttributesFormatString=|
      | %<ID>
      | %<Vbase>V
      | %<VLF>pu
      | %<angleLF>deg.
      | %<Name>
  bus61 : powerlib/Measurements/Load Flow Bus  LConnTagsString=a  ID=bus61  Vbase=132000  Vref=1  Vangle=0  VLF=1  angleLF=0
      settings: AttributesFormatString=|
      | %<ID>
      | %<Vbase>V
      | %<VLF>pu
      | %<angleLF>deg.
      | %<Name>
  bus62 : powerlib/Measurements/Load Flow Bus  LConnTagsString=a  ID=bus62  Vbase=132000  Vref=1  Vangle=0  VLF=1  angleLF=0
      settings: AttributesFormatString=|
      | %<ID>
      | %<Vbase>V
      | %<VLF>pu
      | %<angleLF>deg.
      | %<Name>
  bus63 : powerlib/Measurements/Load Flow Bus  LConnTagsString=a  ID=bus63  Vbase=132000  Vref=1  Vangle=0  VLF=1  angleLF=0
      settings: AttributesFormatString=|
      | %<ID>
      | %<Vbase>V
      | %<VLF>pu
      | %<angleLF>deg.
      | %<Name>
  bus64 : powerlib/Measurements/Load Flow Bus  LConnTagsString=a  ID=bus64  Vbase=132000  Vref=1  Vangle=0  VLF=1  angleLF=0
      settings: AttributesFormatString=|
      | %<ID>
      | %<Vbase>V
      | %<VLF>pu
      | %<angleLF>deg.
      | %<Name>
  bus65 : powerlib/Measurements/Load Flow Bus  LConnTagsString=a  ID=bus65  Vbase=132000  Vref=1  Vangle=0  VLF=1  angleLF=0
      settings: AttributesFormatString=|
      | %<ID>
      | %<Vbase>V
      | %<VLF>pu
      | %<angleLF>deg.
      | %<Name>
  bus66 : powerlib/Measurements/Load Flow Bus  LConnTagsString=a  ID=bus66  Vbase=132000  Vref=1  Vangle=0  VLF=1  angleLF=0
      settings: AttributesFormatString=|
      | %<ID>
      | %<Vbase>V
      | %<VLF>pu
      | %<angleLF>deg.
      | %<Name>
  bus67 : powerlib/Measurements/Load Flow Bus  LConnTagsString=a  ID=bus67  Vbase=132000  Vref=1  Vangle=0  VLF=1  angleLF=0
      settings: AttributesFormatString=|
      | %<ID>
      | %<Vbase>V
      | %<VLF>pu
      | %<angleLF>deg.
      | %<Name>
  bus68 : powerlib/Measurements/Load Flow Bus  LConnTagsString=a  ID=bus68  Vbase=132000  Vref=1  Vangle=0  VLF=1  angleLF=0
      settings: AttributesFormatString=|
      | %<ID>
      | %<Vbase>V
      | %<VLF>pu
      | %<angleLF>deg.
      | %<Name>
  bus69 : powerlib/Measurements/Load Flow Bus  LConnTagsString=a  ID=bus69  Vbase=132000  Vref=1  Vangle=0  VLF=1  angleLF=0
      settings: AttributesFormatString=|
      | %<ID>
      | %<Vbase>V
      | %<VLF>pu
      | %<angleLF>deg.
      | %<Name>
  bus7 : powerlib/Measurements/Load Flow Bus  LConnTagsString=a  ID=bus7  Vbase=50000  Vref=1  Vangle=0  VLF=1  angleLF=0
      settings: AttributesFormatString=|
      | %<ID>
      | %<Vbase>V
      | %<VLF>pu
      | %<angleLF>deg.
      | %<Name>
  bus70 : powerlib/Measurements/Load Flow Bus  LConnTagsString=a  ID=bus70  Vbase=132000  Vref=1  Vangle=0  VLF=1  angleLF=0
      settings: AttributesFormatString=|
      | %<ID>
      | %<Vbase>V
      | %<VLF>pu
      | %<angleLF>deg.
      | %<Name>
  bus71 : powerlib/Measurements/Load Flow Bus  LConnTagsString=a  ID=bus71  Vbase=132000  Vref=1  Vangle=0  VLF=1  angleLF=0
      settings: AttributesFormatString=|
      | %<ID>
      | %<Vbase>V
      | %<VLF>pu
      | %<angleLF>deg.
      | %<Name>
  bus72 : powerlib/Measurements/Load Flow Bus  LConnTagsString=a  ID=bus72  Vbase=132000  Vref=1  Vangle=0  VLF=1  angleLF=0
      settings: AttributesFormatString=|
      | %<ID>
      | %<Vbase>V
      | %<VLF>pu
      | %<angleLF>deg.
      | %<Name>
  bus73 : powerlib/Measurements/Load Flow Bus  LConnTagsString=a  ID=bus73  Vbase=132000  Vref=1  Vangle=0  VLF=1  angleLF=0
      settings: AttributesFormatString=|
      | %<ID>
      | %<Vbase>V
      | %<VLF>pu
      | %<angleLF>deg.
      | %<Name>
  bus74 : powerlib/Measurements/Load Flow Bus  LConnTagsString=a  ID=bus74  Vbase=132000  Vref=1  Vangle=0  VLF=1  angleLF=0
      settings: AttributesFormatString=|
      | %<ID>
      | %<Vbase>V
      | %<VLF>pu
      | %<angleLF>deg.
      | %<Name>
  bus75 : powerlib/Measurements/Load Flow Bus  LConnTagsString=a  ID=bus75  Vbase=132000  Vref=1  Vangle=0  VLF=1  angleLF=0
      settings: AttributesFormatString=|
      | %<ID>
      | %<Vbase>V
      | %<VLF>pu
      | %<angleLF>deg.
      | %<Name>
  bus76 : powerlib/Measurements/Load Flow Bus  LConnTagsString=a  ID=bus76  Vbase=132000  Vref=1  Vangle=0  VLF=1  angleLF=0
      settings: AttributesFormatString=|
      | %<ID>
      | %<Vbase>V
      | %<VLF>pu
      | %<angleLF>deg.
      | %<Name>
  bus77 : powerlib/Measurements/Load Flow Bus  LConnTagsString=a  ID=bus77  Vbase=132000  Vref=1  Vangle=0  VLF=1  angleLF=0
      settings: AttributesFormatString=|
      | %<ID>
      | %<Vbase>V
      | %<VLF>pu
      | %<angleLF>deg.
      | %<Name>
  bus78 : powerlib/Measurements/Load Flow Bus  LConnTagsString=a  ID=bus78  Vbase=132000  Vref=1  Vangle=0  VLF=1  angleLF=0
      settings: AttributesFormatString=|
      | %<ID>
      | %<Vbase>V
      | %<VLF>pu
      | %<angleLF>deg.
      | %<Name>
  bus79 : powerlib/Measurements/Load Flow Bus  LConnTagsString=a  ID=bus79  Vbase=132000  Vref=1  Vangle=0  VLF=1  angleLF=0
      settings: AttributesFormatString=|
      | %<ID>
      | %<Vbase>V
      | %<VLF>pu
      | %<angleLF>deg.
      | %<Name>
  bus8 : powerlib/Measurements/Load Flow Bus  LConnTagsString=a  ID=bus8  Vbase=50000  Vref=1  Vangle=0  VLF=1  angleLF=0
      settings: AttributesFormatString=|
      | %<ID>
      | %<Vbase>V
      | %<VLF>pu
      | %<angleLF>deg.
      | %<Name>
  bus80 : powerlib/Measurements/Load Flow Bus  LConnTagsString=a  ID=bus80  Vbase=132000  Vref=1  Vangle=0  VLF=1  angleLF=0
      settings: AttributesFormatString=|
      | %<ID>
      | %<Vbase>V
      | %<VLF>pu
      | %<angleLF>deg.
      | %<Name>
  bus81 : powerlib/Measurements/Load Flow Bus  LConnTagsString=a  ID=bus81  Vbase=132000  Vref=1  Vangle=0  VLF=1  angleLF=0
      settings: AttributesFormatString=|
      | %<ID>
      | %<Vbase>V
      | %<VLF>pu
      | %<angleLF>deg.
      | %<Name>
  bus82 : powerlib/Measurements/Load Flow Bus  LConnTagsString=a  ID=bus82  Vbase=132000  Vref=1  Vangle=0  VLF=1  angleLF=0
      settings: AttributesFormatString=|
      | %<ID>
      | %<Vbase>V
      | %<VLF>pu
      | %<angleLF>deg.
      | %<Name>
  bus83 : powerlib/Measurements/Load Flow Bus  LConnTagsString=a  ID=bus83  Vbase=132000  Vref=1  Vangle=0  VLF=1  angleLF=0
      settings: AttributesFormatString=|
      | %<ID>
      | %<Vbase>V
      | %<VLF>pu
      | %<angleLF>deg.
      | %<Name>
  bus84 : powerlib/Measurements/Load Flow Bus  LConnTagsString=a  ID=bus84  Vbase=132000  Vref=1  Vangle=0  VLF=1  angleLF=0
      settings: AttributesFormatString=|
      | %<ID>
      | %<Vbase>V
      | %<VLF>pu
      | %<angleLF>deg.
      | %<Name>
  bus85 : powerlib/Measurements/Load Flow Bus  LConnTagsString=a  ID=bus85  Vbase=132000  Vref=1  Vangle=0  VLF=1  angleLF=0
      settings: AttributesFormatString=|
      | %<ID>
      | %<Vbase>V
      | %<VLF>pu
      | %<angleLF>deg.
      | %<Name>
  bus86 : powerlib/Measurements/Load Flow Bus  LConnTagsString=a  ID=bus86  Vbase=132000  Vref=1  Vangle=0  VLF=1  angleLF=0
      settings: AttributesFormatString=|
      | %<ID>
      | %<Vbase>V
      | %<VLF>pu
      | %<angleLF>deg.
      | %<Name>
  bus87 : powerlib/Measurements/Load Flow Bus  LConnTagsString=a  ID=bus87  Vbase=132000  Vref=1  Vangle=0  VLF=1  angleLF=0
      settings: AttributesFormatString=|
      | %<ID>
      | %<Vbase>V
      | %<VLF>pu
      | %<angleLF>deg.
      | %<Name>
  bus88 : powerlib/Measurements/Load Flow Bus  LConnTagsString=a  ID=bus88  Vbase=132000  Vref=1  Vangle=0  VLF=1  angleLF=0
      settings: AttributesFormatString=|
      | %<ID>
      | %<Vbase>V
      | %<VLF>pu
      | %<angleLF>deg.
      | %<Name>
  bus89 : powerlib/Measurements/Load Flow Bus  LConnTagsString=a  ID=bus89  Vbase=132000  Vref=1  Vangle=0  VLF=1  angleLF=0
      settings: AttributesFormatString=|
      | %<ID>
      | %<Vbase>V
      | %<VLF>pu
      | %<angleLF>deg.
      | %<Name>
  bus9 : powerlib/Measurements/Load Flow Bus  LConnTagsString=a  ID=bus9  Vbase=50000  Vref=1  Vangle=0  VLF=1  angleLF=0
      settings: AttributesFormatString=|
      | %<ID>
      | %<Vbase>V
      | %<VLF>pu
      | %<angleLF>deg.
      | %<Name>
  bus90 : powerlib/Measurements/Load Flow Bus  LConnTagsString=a  ID=bus90  Vbase=132000  Vref=1  Vangle=0  VLF=1  angleLF=0
      settings: AttributesFormatString=|
      | %<ID>
      | %<Vbase>V
      | %<VLF>pu
      | %<angleLF>deg.
      | %<Name>
  bus91 : powerlib/Measurements/Load Flow Bus  LConnTagsString=a  ID=bus91  Vbase=132000  Vref=1  Vangle=0  VLF=1  angleLF=0
      settings: AttributesFormatString=|
      | %<ID>
      | %<Vbase>V
      | %<VLF>pu
      | %<angleLF>deg.
      | %<Name>
  bus92 : powerlib/Measurements/Load Flow Bus  LConnTagsString=a  ID=bus92  Vbase=132000  Vref=1  Vangle=0  VLF=1  angleLF=0
      settings: AttributesFormatString=|
      | %<ID>
      | %<Vbase>V
      | %<VLF>pu
      | %<angleLF>deg.
      | %<Name>
  bus93 : powerlib/Measurements/Load Flow Bus  LConnTagsString=a  ID=bus93  Vbase=132000  Vref=1  Vangle=0  VLF=1  angleLF=0
      settings: AttributesFormatString=|
      | %<ID>
      | %<Vbase>V
      | %<VLF>pu
      | %<angleLF>deg.
      | %<Name>
  bus94 : powerlib/Measurements/Load Flow Bus  LConnTagsString=a  ID=bus94  Vbase=132000  Vref=1  Vangle=0  VLF=1  angleLF=0
      settings: AttributesFormatString=|
      | %<ID>
      | %<Vbase>V
      | %<VLF>pu
      | %<angleLF>deg.
      | %<Name>
  bus95 : powerlib/Measurements/Load Flow Bus  LConnTagsString=a  ID=bus95  Vbase=132000  Vref=1  Vangle=0  VLF=1  angleLF=0
      settings: AttributesFormatString=|
      | %<ID>
      | %<Vbase>V
      | %<VLF>pu
      | %<angleLF>deg.
      | %<Name>
  bus96 : powerlib/Measurements/Load Flow Bus  LConnTagsString=a  ID=bus96  Vbase=132000  Vref=1  Vangle=0  VLF=1  angleLF=0
      settings: AttributesFormatString=|
      | %<ID>
      | %<Vbase>V
      | %<VLF>pu
      | %<angleLF>deg.
      | %<Name>
  bus97 : powerlib/Measurements/Load Flow Bus  LConnTagsString=a  ID=bus97  Vbase=132000  Vref=1  Vangle=0  VLF=1  angleLF=0
      settings: AttributesFormatString=|
      | %<ID>
      | %<Vbase>V
      | %<VLF>pu
      | %<angleLF>deg.
      | %<Name>
  bus98 : powerlib/Measurements/Load Flow Bus  LConnTagsString=a  ID=bus98  Vbase=132000  Vref=1  Vangle=0  VLF=1  angleLF=0
      settings: AttributesFormatString=|
      | %<ID>
      | %<Vbase>V
      | %<VLF>pu
      | %<angleLF>deg.
      | %<Name>
  bus99 : powerlib/Measurements/Load Flow Bus  LConnTagsString=a  ID=bus99  Vbase=132000  Vref=1  Vangle=0  VLF=1  angleLF=0
      settings: AttributesFormatString=|
      | %<ID>
      | %<Vbase>V
      | %<VLF>pu
      | %<angleLF>deg.
      | %<Name>
  powergui : powerlib/powergui  Priority=1  SimulationMode=Continuous  SolverType=Tustin  SampleTime=50e-6  frequency=60  SPID=off  DisableSnubberDevices=off  DisableRonSwitches=off  DisableVfSwitches=off  SwTol=0  Interpol=off  DisplayEquations=off  Ts=0  methode=off  frequencyindice=60  Pbase=100e6  ErrMax=1e-4  Iterations=50  UnitsV=kV  UnitsW=MW  FunctionMessages=off  echomessages=off  HookPort=off  EnableUseOfTLC=off  x0status=blocks  RestoreLinks=warning  ResistiveCurrentMeasurement=off  Frange=[0:2:500]  Ylog=off  Xlog=on  ShowGrid=off  save=off  variable=ZData  structure=0  ZoomFFT=off  StartTime=0.0  cycles=1  DisplayStyle=1  fundamental=60  FreqAxis=off  MaxFrequency=1000  frequencyindicesteady=1  RmsSteady=1  display=off
  Åna_Sira_Kjelland_CN_284275993_300000_CN_124861857_300000 : powerlib/Elements/Distributed Parameters Line  Phases=3  Frequency=60  Resistance=[0.01273 0.3864]  Inductance="[0.9337e-3  4.1264e-3]"  Capacitance=[12.74e-9 7.751e-9]  Length=34.0169  x1=[0 0 0 0; 0.0001244 0 0 0; 0.0002488 0 0 0; 0.0003733 0 0 0; 0.0004977 0 0 0; 0.0006221 0 0 0]  x2=[0 0 0 0; 0.0001244 0 0 0; 0.0002488 0 0 0; 0.0003733 0 0 0; 0.0004977 0 0 0; 0.0006221 0 0 0]  x3=[0 0 0 0; 0.0001244 0 0 0; 0.0002488 0 0 0; 0.0003733 0 0 0; 0.0004977 0 0 0; 0.0006221 0 0 0]  x4=[0 0 0 0; 0.0001244 0 0 0; 0.0002488 0 0 0; 0.0003733 0 0 0; 0.0004977 0 0 0; 0.0006221 0 0 0]  x5=0  V1=ones(3,3)  V2=ones(3,3)  I1=ones(3,3)  I2=ones(3,3)  nHarmo=1  Measurements=None
  Ötztal___Zirl_CN_147563007_110000_CN_100404264_110000 : powerlib/Elements/Distributed Parameters Line  Phases=3  Frequency=60  Resistance=[0.01273 0.3864]  Inductance="[0.9337e-3  4.1264e-3]"  Capacitance=[12.74e-9 7.751e-9]  Length=100  x1=[0 0 0 0; 0.0001244 0 0 0; 0.0002488 0 0 0; 0.0003733 0 0 0; 0.0004977 0 0 0; 0.0006221 0 0 0]  x2=[0 0 0 0; 0.0001244 0 0 0; 0.0002488 0 0 0; 0.0003733 0 0 0; 0.0004977 0 0 0; 0.0006221 0 0 0]  x3=[0 0 0 0; 0.0001244 0 0 0; 0.0002488 0 0 0; 0.0003733 0 0 0; 0.0004977 0 0 0; 0.0006221 0 0 0]  x4=[0 0 0 0; 0.0001244 0 0 0; 0.0002488 0 0 0; 0.0003733 0 0 0; 0.0004977 0 0 0; 0.0006221 0 0 0]  x5=0  V1=ones(3,3)  V2=ones(3,3)  I1=ones(3,3)  I2=ones(3,3)  nHarmo=1  Measurements=None
  connections:
  T_288861057__Sande_transformatorstasjon/LConn1 -- Berheim_Sande_1_CN_288861057_50000_CN_166227080_50000/LConn1
  T_288861057__Sande_transformatorstasjon/LConn2 -- Berheim_Sande_1_CN_288861057_50000_CN_166227080_50000/LConn2
  Berheim_Sande_1_CN_288861057_50000_CN_166227080_50000/LConn3 -- T_288861057__Sande_transformatorstasjon/LConn3 -- bus1/LConn1
  Berheim_Sande_1_CN_288861057_50000_CN_166227080_50000/RConn1 -- T_166227080__/RConn1 -- Bærheim_Ulsberget_CN_75805059_50000_CN_166227080_50000/LConn1 -- Berheim_Jåttå_1_CN_166227080_50000_CN_41226817_50000/LConn1 -- Berheim_Skeiane_1_CN_166227080_50000_CN_240212685_50000/LConn1 -- L_166227080/LConn1
  Berheim_Sande_1_CN_288861057_50000_CN_166227080_50000/RConn2 -- T_166227080__/RConn2 -- Bærheim_Ulsberget_CN_75805059_50000_CN_166227080_50000/LConn2 -- Berheim_Jåttå_1_CN_166227080_50000_CN_41226817_50000/LConn2 -- Berheim_Skeiane_1_CN_166227080_50000_CN_240212685_50000/LConn2 -- L_166227080/LConn2
  Berheim_Sande_1_CN_288861057_50000_CN_166227080_50000/RConn3 -- T_166227080__/RConn3 -- Bærheim_Ulsberget_CN_75805059_50000_CN_166227080_50000/LConn3 -- Berheim_Jåttå_1_CN_166227080_50000_CN_41226817_50000/LConn3 -- Berheim_Skeiane_1_CN_166227080_50000_CN_240212685_50000/LConn3 -- L_166227080/LConn3 -- bus2/LConn1
  Forus_Jåttå_CN_75805059_50000_CN_41226817_50000/LConn1 -- T_75805059__Forus_transformatorstasjon/LConn1 -- Bærheim_Ulsberget_CN_75805059_50000_CN_166227080_50000/RConn1
  Forus_Jåttå_CN_75805059_50000_CN_41226817_50000/LConn2 -- T_75805059__Forus_transformatorstasjon/LConn2 -- Bærheim_Ulsberget_CN_75805059_50000_CN_166227080_50000/RConn2
  Forus_Jåttå_CN_75805059_50000_CN_41226817_50000/LConn3 -- T_75805059__Forus_transformatorstasjon/LConn3 -- Bærheim_Ulsberget_CN_75805059_50000_CN_166227080_50000/RConn3 -- bus3/LConn1
  Forus_Jåttå_CN_75805059_50000_CN_41226817_50000/RConn1 -- T_41226817_50000;10000_Jåttå_transformatorstasjon/LConn1 -- Berheim_Jåttå_1_CN_166227080_50000_CN_41226817_50000/RConn1 -- _CN_41226815_50000_CN_41226817_50000/LConn1
  Forus_Jåttå_CN_75805059_50000_CN_41226817_50000/RConn2 -- T_41226817_50000;10000_Jåttå_transformatorstasjon/LConn2 -- Berheim_Jåttå_1_CN_166227080_50000_CN_41226817_50000/RConn2 -- _CN_41226815_50000_CN_41226817_50000/LConn2
  Forus_Jåttå_CN_75805059_50000_CN_41226817_50000/RConn3 -- T_41226817_50000;10000_Jåttå_transformatorstasjon/LConn3 -- Berheim_Jåttå_1_CN_166227080_50000_CN_41226817_50000/RConn3 -- _CN_41226815_50000_CN_41226817_50000/LConn3 -- bus4/LConn1
  Stølaheia_Alsteinsgata_CN_286505477_50000_CN_33793216_50000/LConn1 -- T_286505477_50000_Alsteinsgata_transformatorstasjon/LConn1 -- Kongsgata_Alsteinsgata_CN_286505477_50000_CN_296504285_50000/LConn1
  Stølaheia_Alsteinsgata_CN_286505477_50000_CN_33793216_50000/LConn2 -- T_286505477_50000_Alsteinsgata_transformatorstasjon/LConn2 -- Kongsgata_Alsteinsgata_CN_286505477_50000_CN_296504285_50000/LConn2
  Stølaheia_Alsteinsgata_CN_286505477_50000_CN_33793216_50000/LConn3 -- T_286505477_50000_Alsteinsgata_transformatorstasjon/LConn3 -- Kongsgata_Alsteinsgata_CN_286505477_50000_CN_296504285_50000/LConn3 -- bus5/LConn1
  Stølaheia_Alsteinsgata_CN_286505477_50000_CN_33793216_50000/RConn1 -- T_33793216__Stølaheia_transformatorstasjon/RConn1 -- Stølaheia_Kongsgata_CN_296504285_50000_CN_33793216_50000/LConn1 -- Stølaheia_Madla_1_CN_36163257_50000_CN_33793216_50000/LConn1 -- Stølaheia_Randaberg_1_CN_33793216_50000_CN_139346918_50000/LConn1 -- Stølaheia_Båtstad_CN_33793216_50000_CN_297123048_50000/LConn1 -- L_33793216/LConn1
  Stølaheia_Alsteinsgata_CN_286505477_50000_CN_33793216_50000/RConn2 -- T_33793216__Stølaheia_transformatorstasjon/RConn2 -- Stølaheia_Kongsgata_CN_296504285_50000_CN_33793216_50000/LConn2 -- Stølaheia_Madla_1_CN_36163257_50000_CN_33793216_50000/LConn2 -- Stølaheia_Randaberg_1_CN_33793216_50000_CN_139346918_50000/LConn2 -- Stølaheia_Båtstad_CN_33793216_50000_CN_297123048_50000/LConn2 -- L_33793216/LConn2
  Stølaheia_Alsteinsgata_CN_286505477_50000_CN_33793216_50000/RConn3 -- T_33793216__Stølaheia_transformatorstasjon/RConn3 -- Stølaheia_Kongsgata_CN_296504285_50000_CN_33793216_50000/LConn3 -- Stølaheia_Madla_1_CN_36163257_50000_CN_33793216_50000/LConn3 -- Stølaheia_Randaberg_1_CN_33793216_50000_CN_139346918_50000/LConn3 -- Stølaheia_Båtstad_CN_33793216_50000_CN_297123048_50000/LConn3 -- L_33793216/LConn3 -- bus6/LConn1
  Kongsgata_Alsteinsgata_CN_286505477_50000_CN_296504285_50000/RConn1 -- T_296504285__Kongsgata/LConn1 -- Mosvannet_Kongsgt_CN_296504285_50000_CN_91655624_50000/LConn1 -- Stølaheia_Kongsgata_CN_296504285_50000_CN_33793216_50000/RConn1
  Kongsgata_Alsteinsgata_CN_286505477_50000_CN_296504285_50000/RConn2 -- T_296504285__Kongsgata/LConn2 -- Mosvannet_Kongsgt_CN_296504285_50000_CN_91655624_50000/LConn2 -- Stølaheia_Kongsgata_CN_296504285_50000_CN_33793216_50000/RConn2
  Kongsgata_Alsteinsgata_CN_286505477_50000_CN_296504285_50000/RConn3 -- T_296504285__Kongsgata/LConn3 -- Mosvannet_Kongsgt_CN_296504285_50000_CN_91655624_50000/LConn3 -- Stølaheia_Kongsgata_CN_296504285_50000_CN_33793216_50000/RConn3 -- bus7/LConn1
  T_240212685_50000_Lura_transformatorstasjon/LConn1 -- Berheim_Skeiane_1_CN_166227080_50000_CN_240212685_50000/RConn1
  T_240212685_50000_Lura_transformatorstasjon/LConn2 -- Berheim_Skeiane_1_CN_166227080_50000_CN_240212685_50000/RConn2
  Berheim_Skeiane_1_CN_166227080_50000_CN_240212685_50000/RConn3 -- T_240212685_50000_Lura_transformatorstasjon/LConn3 -- bus8/LConn1
  Nærbø_Opstad_CN_284260110_50000_CN_329581844_50000/LConn1 -- T_284260110_50000;22000_Opstad_trafostasjon/LConn1 -- Opstad_(Bø)_Hetland_CN_284260110_50000_CN_285825522_50000/LConn1 -- Holen_Opstad_CN_284260110_50000_CN_290983494_50000/LConn1
  Nærbø_Opstad_CN_284260110_50000_CN_329581844_50000/LConn2 -- T_284260110_50000;22000_Opstad_trafostasjon/LConn2 -- Opstad_(Bø)_Hetland_CN_284260110_50000_CN_285825522_50000/LConn2 -- Holen_Opstad_CN_284260110_50000_CN_290983494_50000/LConn2
  Nærbø_Opstad_CN_284260110_50000_CN_329581844_50000/LConn3 -- T_284260110_50000;22000_Opstad_trafostasjon/LConn3 -- Opstad_(Bø)_Hetland_CN_284260110_50000_CN_285825522_50000/LConn3 -- Holen_Opstad_CN_284260110_50000_CN_290983494_50000/LConn3 -- bus9/LConn1
  Nærbø_Opstad_CN_284260110_50000_CN_329581844_50000/RConn1 -- T_329581844_50000;medium_Nærbø_transformatorstasjon/LConn1 -- Nærbø_Håland_CN_329581844_50000_CN_285809906_50000/LConn1
  Nærbø_Opstad_CN_284260110_50000_CN_329581844_50000/RConn2 -- T_329581844_50000;medium_Nærbø_transformatorstasjon/LConn2 -- Nærbø_Håland_CN_329581844_50000_CN_285809906_50000/LConn2
  Nærbø_Opstad_CN_284260110_50000_CN_329581844_50000/RConn3 -- T_329581844_50000;medium_Nærbø_transformatorstasjon/LConn3 -- Nærbø_Håland_CN_329581844_50000_CN_285809906_50000/LConn3 -- bus10/LConn1
  G_285825522_Hetland_kraftverk/RConn1 -- Opstad_(Bø)_Hetland_CN_284260110_50000_CN_285825522_50000/RConn1
  G_285825522_Hetland_kraftverk/RConn2 -- Opstad_(Bø)_Hetland_CN_284260110_50000_CN_285825522_50000/RConn2
  Opstad_(Bø)_Hetland_CN_284260110_50000_CN_285825522_50000/RConn3 -- G_285825522_Hetland_kraftverk/RConn3 -- bus11/LConn1
  Holen_Opstad_CN_284260110_50000_CN_290983494_50000/RConn1 -- T_290983494__/LConn1 -- Vagle_Kalberg_1_CN_329581840_50000_CN_290983494_50000/LConn1 -- Holen_Håland_CN_290983494_50000_CN_285809906_50000/LConn1 -- _CN_290983494_50000_CN_285976807_50000/LConn1
  Holen_Opstad_CN_284260110_50000_CN_290983494_50000/RConn2 -- T_290983494__/LConn2 -- Vagle_Kalberg_1_CN_329581840_50000_CN_290983494_50000/LConn2 -- Holen_Håland_CN_290983494_50000_CN_285809906_50000/LConn2 -- _CN_290983494_50000_CN_285976807_50000/LConn2
  Holen_Opstad_CN_284260110_50000_CN_290983494_50000/RConn3 -- T_290983494__/LConn3 -- Vagle_Kalberg_1_CN_329581840_50000_CN_290983494_50000/LConn3 -- Holen_Håland_CN_290983494_50000_CN_285809906_50000/LConn3 -- _CN_290983494_50000_CN_285976807_50000/LConn3 -- bus12/LConn1
  Vagle_Kalberg_1_CN_329581840_50000_CN_290983494_50000/RConn1 -- T_329581840__Kalberg_transformatorstasjon/LConn1 -- Vagle_Kalberg_1_CN_329581840_50000_CN_284251750_50000/LConn1
  Vagle_Kalberg_1_CN_329581840_50000_CN_290983494_50000/RConn2 -- T_329581840__Kalberg_transformatorstasjon/LConn2 -- Vagle_Kalberg_1_CN_329581840_50000_CN_284251750_50000/LConn2
  Vagle_Kalberg_1_CN_329581840_50000_CN_290983494_50000/RConn3 -- T_329581840__Kalberg_transformatorstasjon/LConn3 -- Vagle_Kalberg_1_CN_329581840_50000_CN_284251750_50000/LConn3 -- bus13/LConn1
  Vagle_Kalberg_1_CN_329581840_50000_CN_284251750_50000/RConn1 -- T_284251750__Vagle_transformatorstasjon/LConn1 -- Vagle_Hatteland_1_CN_284251750_50000_CN_285809905_50000/LConn1 -- Tronsholen_Vagle_2_CN_284251750_50000_CN_50192634_50000/LConn1
  Vagle_Kalberg_1_CN_329581840_50000_CN_284251750_50000/RConn2 -- T_284251750__Vagle_transformatorstasjon/LConn2 -- Vagle_Hatteland_1_CN_284251750_50000_CN_285809905_50000/LConn2 -- Tronsholen_Vagle_2_CN_284251750_50000_CN_50192634_50000/LConn2
  Vagle_Kalberg_1_CN_329581840_50000_CN_284251750_50000/RConn3 -- T_284251750__Vagle_transformatorstasjon/LConn3 -- Vagle_Hatteland_1_CN_284251750_50000_CN_285809905_50000/LConn3 -- Tronsholen_Vagle_2_CN_284251750_50000_CN_50192634_50000/LConn3 -- bus14/LConn1
  Nærbø_Håland_CN_329581844_50000_CN_285809906_50000/RConn1 -- T_285809906__Håland_trafostasjon/LConn1 -- Holen_Håland_CN_290983494_50000_CN_285809906_50000/RConn1
  Nærbø_Håland_CN_329581844_50000_CN_285809906_50000/RConn2 -- T_285809906__Håland_trafostasjon/LConn2 -- Holen_Håland_CN_290983494_50000_CN_285809906_50000/RConn2
  Nærbø_Håland_CN_329581844_50000_CN_285809906_50000/RConn3 -- T_285809906__Håland_trafostasjon/LConn3 -- Holen_Håland_CN_290983494_50000_CN_285809906_50000/RConn3 -- bus15/LConn1
  T_89032743__Hillevåg_transformatorstasjon/LConn1 -- Ullandhaug_Hillevåg_CN_89032743_50000_CN_41226815_50000/LConn1
  T_89032743__Hillevåg_transformatorstasjon/LConn2 -- Ullandhaug_Hillevåg_CN_89032743_50000_CN_41226815_50000/LConn2
  Ullandhaug_Hillevåg_CN_89032743_50000_CN_41226815_50000/LConn3 -- T_89032743__Hillevåg_transformatorstasjon/LConn3 -- bus16/LConn1
  Ullandhaug_Hillevåg_CN_89032743_50000_CN_41226815_50000/RConn1 -- T_41226815__Ullandhaug_transformatorstasjon/LConn1 -- Ullandhaug_Tjensvoll_2_CN_96439090_50000_CN_41226815_50000/LConn1 -- Ullandhaug_Haugesundsgata_CN_41226815_50000_CN_289487098_50000/LConn1 -- _CN_41226815_50000_CN_41226817_50000/RConn1 -- _CN_41226815_50000_CN_91655624_50000/LConn1
  Ullandhaug_Hillevåg_CN_89032743_50000_CN_41226815_50000/RConn2 -- T_41226815__Ullandhaug_transformatorstasjon/LConn2 -- Ullandhaug_Tjensvoll_2_CN_96439090_50000_CN_41226815_50000/LConn2 -- Ullandhaug_Haugesundsgata_CN_41226815_50000_CN_289487098_50000/LConn2 -- _CN_41226815_50000_CN_41226817_50000/RConn2 -- _CN_41226815_50000_CN_91655624_50000/LConn2
  Ullandhaug_Hillevåg_CN_89032743_50000_CN_41226815_50000/RConn3 -- T_41226815__Ullandhaug_transformatorstasjon/LConn3 -- Ullandhaug_Tjensvoll_2_CN_96439090_50000_CN_41226815_50000/LConn3 -- Ullandhaug_Haugesundsgata_CN_41226815_50000_CN_289487098_50000/LConn3 -- _CN_41226815_50000_CN_41226817_50000/RConn3 -- _CN_41226815_50000_CN_91655624_50000/LConn3 -- bus17/LConn1
  T_112412584__Vatne_transformatorstasjon/LConn1 -- Vatne_Riska_CN_112412584_50000_CN_329592517_50000/LConn1
  T_112412584__Vatne_transformatorstasjon/LConn2 -- Vatne_Riska_CN_112412584_50000_CN_329592517_50000/LConn2
  Vatne_Riska_CN_112412584_50000_CN_329592517_50000/LConn3 -- T_112412584__Vatne_transformatorstasjon/LConn3 -- bus18/LConn1
  Vatne_Riska_CN_112412584_50000_CN_329592517_50000/RConn1 -- T_329592517_50000;medium_Riska_transformatorstasjon/LConn1 -- Oltedal_Riska_CN_329592517_50000_CN_297122914_50000/LConn1
  Vatne_Riska_CN_112412584_50000_CN_329592517_50000/RConn2 -- T_329592517_50000;medium_Riska_transformatorstasjon/LConn2 -- Oltedal_Riska_CN_329592517_50000_CN_297122914_50000/LConn2
  Vatne_Riska_CN_112412584_50000_CN_329592517_50000/RConn3 -- T_329592517_50000;medium_Riska_transformatorstasjon/LConn3 -- Oltedal_Riska_CN_329592517_50000_CN_297122914_50000/LConn3 -- bus19/LConn1
  Dusavik_Buøy_CN_295444551_50000_CN_139346918_50000/LConn1 -- T_295444551__Buøy_transformatorstasjon/LConn1 -- Haugesundsgata_Buøy_CN_295444551_50000_CN_289487098_50000/LConn1
  Dusavik_Buøy_CN_295444551_50000_CN_139346918_50000/LConn2 -- T_295444551__Buøy_transformatorstasjon/LConn2 -- Haugesundsgata_Buøy_CN_295444551_50000_CN_289487098_50000/LConn2
  Dusavik_Buøy_CN_295444551_50000_CN_139346918_50000/LConn3 -- T_295444551__Buøy_transformatorstasjon/LConn3 -- Haugesundsgata_Buøy_CN_295444551_50000_CN_289487098_50000/LConn3 -- bus20/LConn1
  Dusavik_Buøy_CN_295444551_50000_CN_139346918_50000/RConn1 -- T_139346918_50000_Dusavik/LConn1 -- Stølaheia_Randaberg_1_CN_33793216_50000_CN_139346918_50000/RConn1
  Dusavik_Buøy_CN_295444551_50000_CN_139346918_50000/RConn2 -- T_139346918_50000_Dusavik/LConn2 -- Stølaheia_Randaberg_1_CN_33793216_50000_CN_139346918_50000/RConn2
  Dusavik_Buøy_CN_295444551_50000_CN_139346918_50000/RConn3 -- T_139346918_50000_Dusavik/LConn3 -- Stølaheia_Randaberg_1_CN_33793216_50000_CN_139346918_50000/RConn3 -- bus21/LConn1
  Haugesundsgata_Buøy_CN_295444551_50000_CN_289487098_50000/RConn1 -- T_289487098__Haugesundsgata_transformatorstasjon/LConn1 -- Ullandhaug_Haugesundsgata_CN_41226815_50000_CN_289487098_50000/RConn1
  Haugesundsgata_Buøy_CN_295444551_50000_CN_289487098_50000/RConn2 -- T_289487098__Haugesundsgata_transformatorstasjon/LConn2 -- Ullandhaug_Haugesundsgata_CN_41226815_50000_CN_289487098_50000/RConn2
  Haugesundsgata_Buøy_CN_295444551_50000_CN_289487098_50000/RConn3 -- T_289487098__Haugesundsgata_transformatorstasjon/LConn3 -- Ullandhaug_Haugesundsgata_CN_41226815_50000_CN_289487098_50000/RConn3 -- bus22/LConn1
  Mosvannet_Kongsgt_CN_296504285_50000_CN_91655624_50000/RConn1 -- T_91655624__/LConn1 -- _CN_41226815_50000_CN_91655624_50000/RConn1
  Mosvannet_Kongsgt_CN_296504285_50000_CN_91655624_50000/RConn2 -- T_91655624__/LConn2 -- _CN_41226815_50000_CN_91655624_50000/RConn2
  Mosvannet_Kongsgt_CN_296504285_50000_CN_91655624_50000/RConn3 -- T_91655624__/LConn3 -- _CN_41226815_50000_CN_91655624_50000/RConn3 -- bus23/LConn1
  T_96439090__/LConn1 -- Ullandhaug_Tjensvoll_2_CN_96439090_50000_CN_41226815_50000/RConn1
  T_96439090__/LConn2 -- Ullandhaug_Tjensvoll_2_CN_96439090_50000_CN_41226815_50000/RConn2
  Ullandhaug_Tjensvoll_2_CN_96439090_50000_CN_41226815_50000/RConn3 -- T_96439090__/LConn3 -- bus24/LConn1
  T_36163257__/LConn1 -- Stølaheia_Madla_1_CN_36163257_50000_CN_33793216_50000/RConn1
  T_36163257__/LConn2 -- Stølaheia_Madla_1_CN_36163257_50000_CN_33793216_50000/RConn2
  Stølaheia_Madla_1_CN_36163257_50000_CN_33793216_50000/RConn3 -- T_36163257__/LConn3 -- bus25/LConn1
  HVDC_Cross_Skagerak_CN_287687994_50000_CN_129017290_50000/LConn1 -- T_287687994_420000;300000_/RConn4 -- L_287687994/LConn1
  HVDC_Cross_Skagerak_CN_287687994_50000_CN_129017290_50000/LConn2 -- T_287687994_420000;300000_/RConn5 -- L_287687994/LConn2
  HVDC_Cross_Skagerak_CN_287687994_50000_CN_129017290_50000/LConn3 -- T_287687994_420000;300000_/RConn6 -- L_287687994/LConn3 -- bus26/LConn1
  T_129017290__/LConn1 -- HVDC_Cross_Skagerak_CN_287687994_50000_CN_129017290_50000/RConn1
  T_129017290__/LConn2 -- HVDC_Cross_Skagerak_CN_287687994_50000_CN_129017290_50000/RConn2
  HVDC_Cross_Skagerak_CN_287687994_50000_CN_129017290_50000/RConn3 -- T_129017290__/LConn3 -- bus27/LConn1
  T_297123048_50000_Båtstad_transformatorstasjon/LConn1 -- Stølaheia_Båtstad_CN_33793216_50000_CN_297123048_50000/RConn1
  T_297123048_50000_Båtstad_transformatorstasjon/LConn2 -- Stølaheia_Båtstad_CN_33793216_50000_CN_297123048_50000/RConn2
  Stølaheia_Båtstad_CN_33793216_50000_CN_297123048_50000/RConn3 -- T_297123048_50000_Båtstad_transformatorstasjon/LConn3 -- bus28/LConn1
  T_297122914__Ålgård_transformatorstasjon/LConn1 -- Oltedal_Riska_CN_329592517_50000_CN_297122914_50000/RConn1
  T_297122914__Ålgård_transformatorstasjon/LConn2 -- Oltedal_Riska_CN_329592517_50000_CN_297122914_50000/RConn2
  Oltedal_Riska_CN_329592517_50000_CN_297122914_50000/RConn3 -- T_297122914__Ålgård_transformatorstasjon/LConn3 -- bus29/LConn1
  _CN_290983494_50000_CN_285976807_50000/RConn1 -- T_285976807__Tu_trafostasjon/LConn1 -- Hatteland_Tu_CN_285976807_50000_CN_285809905_50000/LConn1
  _CN_290983494_50000_CN_285976807_50000/RConn2 -- T_285976807__Tu_trafostasjon/LConn2 -- Hatteland_Tu_CN_285976807_50000_CN_285809905_50000/LConn2
  _CN_290983494_50000_CN_285976807_50000/RConn3 -- T_285976807__Tu_trafostasjon/LConn3 -- Hatteland_Tu_CN_285976807_50000_CN_285809905_50000/LConn3 -- bus30/LConn1
  Vagle_Hatteland_1_CN_284251750_50000_CN_285809905_50000/RConn1 -- T_285809905__Hatteland_trafostasjon/LConn1 -- _CN_290896873_50000_CN_285809905_50000/LConn1 -- Hatteland_Tu_CN_285976807_50000_CN_285809905_50000/RConn1
  Vagle_Hatteland_1_CN_284251750_50000_CN_285809905_50000/RConn2 -- T_285809905__Hatteland_trafostasjon/LConn2 -- _CN_290896873_50000_CN_285809905_50000/LConn2 -- Hatteland_Tu_CN_285976807_50000_CN_285809905_50000/RConn2
  Vagle_Hatteland_1_CN_284251750_50000_CN_285809905_50000/RConn3 -- T_285809905__Hatteland_trafostasjon/LConn3 -- _CN_290896873_50000_CN_285809905_50000/LConn3 -- bus31/LConn1 -- Hatteland_Tu_CN_285976807_50000_CN_285809905_50000/RConn3
  Tronsholen_Vagle_2_CN_284251750_50000_CN_50192634_50000/RConn1 -- T_50192634__Tronsholen/RConn1 -- L_50192634/LConn1
  Tronsholen_Vagle_2_CN_284251750_50000_CN_50192634_50000/RConn2 -- T_50192634__Tronsholen/RConn2 -- L_50192634/LConn2
  Tronsholen_Vagle_2_CN_284251750_50000_CN_50192634_50000/RConn3 -- T_50192634__Tronsholen/RConn3 -- L_50192634/LConn3 -- bus32/LConn1
  T_290896873__Kleppemarka_trafostasjon/LConn1 -- _CN_290896873_50000_CN_285809905_50000/RConn1
  T_290896873__Kleppemarka_trafostasjon/LConn2 -- _CN_290896873_50000_CN_285809905_50000/RConn2
  _CN_290896873_50000_CN_285809905_50000/RConn3 -- T_290896873__Kleppemarka_trafostasjon/LConn3 -- bus33/LConn1
  _CN_295444099_66000_CN_384765294_66000/LConn1 -- T_295444099_420000;300000;66000_Frogner_transformatorstasjon/RConn4 -- _CN_295444099_66000_CN_88729162_66000/LConn1 -- _CN_295444099_66000_CN_295444119_66000/LConn1 -- _CN_295444099_66000_CN_92116523_66000/LConn1 -- Frogner_Gjestad_1&2_CN_295444099_66000_CN_295444109_66000/LConn1 -- L_295444099/LConn1 -- _CN_295444099_66000_CN_118272324_66000/LConn1
  _CN_295444099_66000_CN_384765294_66000/LConn2 -- T_295444099_420000;300000;66000_Frogner_transformatorstasjon/RConn5 -- _CN_295444099_66000_CN_88729162_66000/LConn2 -- _CN_295444099_66000_CN_295444119_66000/LConn2 -- _CN_295444099_66000_CN_92116523_66000/LConn2 -- Frogner_Gjestad_1&2_CN_295444099_66000_CN_295444109_66000/LConn2 -- L_295444099/LConn2 -- _CN_295444099_66000_CN_118272324_66000/LConn2
  _CN_295444099_66000_CN_384765294_66000/LConn3 -- T_295444099_420000;300000;66000_Frogner_transformatorstasjon/RConn6 -- _CN_295444099_66000_CN_88729162_66000/LConn3 -- _CN_295444099_66000_CN_295444119_66000/LConn3 -- _CN_295444099_66000_CN_92116523_66000/LConn3 -- Frogner_Gjestad_1&2_CN_295444099_66000_CN_295444109_66000/LConn3 -- L_295444099/LConn3 -- bus34/LConn1 -- _CN_295444099_66000_CN_118272324_66000/LConn3
  _CN_295444099_66000_CN_384765294_66000/RConn1 -- T_384765294__/LConn1 -- _CN_384765294_66000_CN_384765297_66000/LConn1
  _CN_295444099_66000_CN_384765294_66000/RConn2 -- T_384765294__/LConn2 -- _CN_384765294_66000_CN_384765297_66000/LConn2
  _CN_295444099_66000_CN_384765294_66000/RConn3 -- T_384765294__/LConn3 -- _CN_384765294_66000_CN_384765297_66000/LConn3 -- bus35/LConn1
  _CN_295444099_66000_CN_118272324_66000/RConn1 -- T_118272324_66000_Nerdrum_transformator/LConn1 -- Nerdrum_1_CN_113574844_66000_CN_118272324_66000/LConn1
  _CN_295444099_66000_CN_118272324_66000/RConn2 -- T_118272324_66000_Nerdrum_transformator/LConn2 -- Nerdrum_1_CN_113574844_66000_CN_118272324_66000/LConn2
  _CN_295444099_66000_CN_118272324_66000/RConn3 -- T_118272324_66000_Nerdrum_transformator/LConn3 -- Nerdrum_1_CN_113574844_66000_CN_118272324_66000/LConn3 -- bus36/LConn1
  _CN_295444099_66000_CN_88729162_66000/RConn1 -- T_88729162_66000_?_transformatorstasjon/LConn1 -- Kjellerholen_1&2_CN_88729162_66000_CN_48798062_66000/LConn1 -- Nerdrum_1_CN_113574844_66000_CN_88729162_66000/LConn1
  _CN_295444099_66000_CN_88729162_66000/RConn2 -- T_88729162_66000_?_transformatorstasjon/LConn2 -- Kjellerholen_1&2_CN_88729162_66000_CN_48798062_66000/LConn2 -- Nerdrum_1_CN_113574844_66000_CN_88729162_66000/LConn2
  _CN_295444099_66000_CN_88729162_66000/RConn3 -- T_88729162_66000_?_transformatorstasjon/LConn3 -- Kjellerholen_1&2_CN_88729162_66000_CN_48798062_66000/LConn3 -- bus37/LConn1 -- Nerdrum_1_CN_113574844_66000_CN_88729162_66000/LConn3
  T_295444119__Vestbygata_transformatorstasjon/LConn1 -- _CN_295444099_66000_CN_295444119_66000/RConn1
  T_295444119__Vestbygata_transformatorstasjon/LConn2 -- _CN_295444099_66000_CN_295444119_66000/RConn2
  _CN_295444099_66000_CN_295444119_66000/RConn3 -- T_295444119__Vestbygata_transformatorstasjon/LConn3 -- bus38/LConn1
  T_92116523__Strøm_transformatorstasjon/LConn1 -- _CN_295444099_66000_CN_92116523_66000/RConn1
  T_92116523__Strøm_transformatorstasjon/LConn2 -- _CN_295444099_66000_CN_92116523_66000/RConn2
  _CN_295444099_66000_CN_92116523_66000/RConn3 -- T_92116523__Strøm_transformatorstasjon/LConn3 -- bus39/LConn1
  T_295444109__Gjestad_transformatorstasjon/LConn1 -- Frogner_Gjestad_1&2_CN_295444099_66000_CN_295444109_66000/RConn1
  T_295444109__Gjestad_transformatorstasjon/LConn2 -- Frogner_Gjestad_1&2_CN_295444099_66000_CN_295444109_66000/RConn2
  Frogner_Gjestad_1&2_CN_295444099_66000_CN_295444109_66000/RConn3 -- T_295444109__Gjestad_transformatorstasjon/LConn3 -- bus40/LConn1
  T_98937735__/LConn1 -- _CN_98937735_66000_CN_185427154_66000/LConn1
  T_98937735__/LConn2 -- _CN_98937735_66000_CN_185427154_66000/LConn2
  _CN_98937735_66000_CN_185427154_66000/LConn3 -- T_98937735__/LConn3 -- bus41/LConn1
  _CN_98937735_66000_CN_185427154_66000/RConn1 -- T_185427154__/LConn1 -- _CN_60495669_66000_CN_185427154_66000/LConn1
  _CN_98937735_66000_CN_185427154_66000/RConn2 -- T_185427154__/LConn2 -- _CN_60495669_66000_CN_185427154_66000/LConn2
  _CN_98937735_66000_CN_185427154_66000/RConn3 -- T_185427154__/LConn3 -- _CN_60495669_66000_CN_185427154_66000/LConn3 -- bus42/LConn1
  T_384765297__Løken_transformator/LConn1 -- _CN_384765294_66000_CN_384765297_66000/RConn1
  T_384765297__Løken_transformator/LConn2 -- _CN_384765294_66000_CN_384765297_66000/RConn2
  _CN_384765294_66000_CN_384765297_66000/RConn3 -- T_384765297__Løken_transformator/LConn3 -- bus43/LConn1
  T_90078235__/LConn1 -- _CN_90078235_66000_CN_114336709_66000/LConn1
  T_90078235__/LConn2 -- _CN_90078235_66000_CN_114336709_66000/LConn2
  _CN_90078235_66000_CN_114336709_66000/LConn3 -- T_90078235__/LConn3 -- bus44/LConn1
  _CN_90078235_66000_CN_114336709_66000/RConn1 -- T_114336709_300000;132000_Vang_trafostasjon/RConn4 -- L_114336709/LConn1
  _CN_90078235_66000_CN_114336709_66000/RConn2 -- T_114336709_300000;132000_Vang_trafostasjon/RConn5 -- L_114336709/LConn2
  _CN_90078235_66000_CN_114336709_66000/RConn3 -- T_114336709_300000;132000_Vang_trafostasjon/RConn6 -- L_114336709/LConn3 -- bus45/LConn1
  _CN_60495669_66000_CN_185427154_66000/RConn1 -- T_60495669_420000;300000;132000_Hasle_Transformatorstasjon/RConn1 -- L_60495669/LConn1
  _CN_60495669_66000_CN_185427154_66000/RConn2 -- T_60495669_420000;300000;132000_Hasle_Transformatorstasjon/RConn2 -- L_60495669/LConn2
  _CN_60495669_66000_CN_185427154_66000/RConn3 -- T_60495669_420000;300000;132000_Hasle_Transformatorstasjon/RConn3 -- L_60495669/LConn3 -- bus46/LConn1
  Nerdrum_1_CN_113574844_66000_CN_88729162_66000/RConn1 -- T_113574844__/LConn1 -- Nerdrum_1_CN_113574844_66000_CN_118272324_66000/RConn1
  Nerdrum_1_CN_113574844_66000_CN_88729162_66000/RConn2 -- T_113574844__/LConn2 -- Nerdrum_1_CN_113574844_66000_CN_118272324_66000/RConn2
  Nerdrum_1_CN_113574844_66000_CN_88729162_66000/RConn3 -- T_113574844__/LConn3 -- Nerdrum_1_CN_113574844_66000_CN_118272324_66000/RConn3 -- bus47/LConn1
  Kjellerholen_1&2_CN_88729162_66000_CN_48798062_66000/RConn1 -- T_48798062_300000_Røykås_trafostasjon/RConn1 -- L_48798062/LConn1
  Kjellerholen_1&2_CN_88729162_66000_CN_48798062_66000/RConn2 -- T_48798062_300000_Røykås_trafostasjon/RConn2 -- L_48798062/LConn2
  Kjellerholen_1&2_CN_88729162_66000_CN_48798062_66000/RConn3 -- T_48798062_300000_Røykås_trafostasjon/RConn3 -- L_48798062/LConn3 -- bus48/LConn1
  T_90139980__/LConn1 -- _CN_90139980_66000_CN_106879472_66000/LConn1
  T_90139980__/LConn2 -- _CN_90139980_66000_CN_106879472_66000/LConn2
  _CN_90139980_66000_CN_106879472_66000/LConn3 -- T_90139980__/LConn3 -- bus49/LConn1
  T_106879472__/LConn1 -- _CN_90139980_66000_CN_106879472_66000/RConn1
  T_106879472__/LConn2 -- _CN_90139980_66000_CN_106879472_66000/RConn2
  _CN_90139980_66000_CN_106879472_66000/RConn3 -- T_106879472__/LConn3 -- bus50/LConn1
  T_202200064_132000_Aura/LConn1 -- _CN_202200064_132000_CN_202200068_132000/LConn1
  T_202200064_132000_Aura/LConn2 -- _CN_202200064_132000_CN_202200068_132000/LConn2
  _CN_202200064_132000_CN_202200068_132000/LConn3 -- T_202200064_132000_Aura/LConn3 -- bus51/LConn1
  _CN_202200064_132000_CN_202200068_132000/RConn1 -- T_202200068_132000_/LConn1 -- _CN_202200066_132000_CN_202200068_132000/LConn1
  _CN_202200064_132000_CN_202200068_132000/RConn2 -- T_202200068_132000_/LConn2 -- _CN_202200066_132000_CN_202200068_132000/LConn2
  _CN_202200064_132000_CN_202200068_132000/RConn3 -- T_202200068_132000_/LConn3 -- _CN_202200066_132000_CN_202200068_132000/LConn3 -- bus52/LConn1
  _CN_202200066_132000_CN_202200068_132000/RConn1 -- T_202200066_420000;132000_Viklandet/RConn1 -- L_202200066/LConn1
  _CN_202200066_132000_CN_202200068_132000/RConn2 -- T_202200066_420000;132000_Viklandet/RConn2 -- L_202200066/LConn2
  _CN_202200066_132000_CN_202200068_132000/RConn3 -- T_202200066_420000;132000_Viklandet/RConn3 -- L_202200066/LConn3 -- bus53/LConn1
  T_432917507__/LConn1 -- _CN_432917507_132000_CN_333991713_132000/LConn1
  T_432917507__/LConn2 -- _CN_432917507_132000_CN_333991713_132000/LConn2
  _CN_432917507_132000_CN_333991713_132000/LConn3 -- T_432917507__/LConn3 -- bus54/LConn1
  _CN_432917507_132000_CN_333991713_132000/RConn1 -- T_333991713__Fana_transformatorstasjon/RConn1 -- _CN_401860888_132000_CN_333991713_132000/LConn1 -- L_333991713/LConn1
  _CN_432917507_132000_CN_333991713_132000/RConn2 -- T_333991713__Fana_transformatorstasjon/RConn2 -- _CN_401860888_132000_CN_333991713_132000/LConn2 -- L_333991713/LConn2
  _CN_432917507_132000_CN_333991713_132000/RConn3 -- T_333991713__Fana_transformatorstasjon/RConn3 -- _CN_401860888_132000_CN_333991713_132000/LConn3 -- L_333991713/LConn3 -- bus55/LConn1
  T_92630533_132000_/LConn1 -- _CN_92630533_132000_CN_92630638_132000/LConn1
  T_92630533_132000_/LConn2 -- _CN_92630533_132000_CN_92630638_132000/LConn2
  _CN_92630533_132000_CN_92630638_132000/LConn3 -- T_92630533_132000_/LConn3 -- bus56/LConn1
  G_92630638_/RConn1 -- _CN_92630533_132000_CN_92630638_132000/RConn1
  G_92630638_/RConn2 -- _CN_92630533_132000_CN_92630638_132000/RConn2
  _CN_92630533_132000_CN_92630638_132000/RConn3 -- G_92630638_/RConn3 -- bus57/LConn1
  T_26938543_132000_/LConn1 -- _CN_26938543_132000_CN_27030901_132000/LConn1
  T_26938543_132000_/LConn2 -- _CN_26938543_132000_CN_27030901_132000/LConn2
  _CN_26938543_132000_CN_27030901_132000/LConn3 -- T_26938543_132000_/LConn3 -- bus58/LConn1
  T_27030901_132000_/LConn1 -- _CN_26938543_132000_CN_27030901_132000/RConn1
  T_27030901_132000_/LConn2 -- _CN_26938543_132000_CN_27030901_132000/RConn2
  _CN_26938543_132000_CN_27030901_132000/RConn3 -- T_27030901_132000_/LConn3 -- bus59/LConn1
  T_355844785__/LConn1 -- _CN_355844785_132000_CN_355844774_132000/LConn1
  T_355844785__/LConn2 -- _CN_355844785_132000_CN_355844774_132000/LConn2
  _CN_355844785_132000_CN_355844774_132000/LConn3 -- T_355844785__/LConn3 -- bus60/LConn1
  T_355844774__/LConn1 -- _CN_355844785_132000_CN_355844774_132000/RConn1
  T_355844774__/LConn2 -- _CN_355844785_132000_CN_355844774_132000/RConn2
  _CN_355844785_132000_CN_355844774_132000/RConn3 -- T_355844774__/LConn3 -- bus61/LConn1
  T_111859753__/LConn1 -- _CN_111859753_132000_CN_103088765_132000/LConn1
  T_111859753__/LConn2 -- _CN_111859753_132000_CN_103088765_132000/LConn2
  _CN_111859753_132000_CN_103088765_132000/LConn3 -- T_111859753__/LConn3 -- bus62/LConn1
  _CN_111859753_132000_CN_103088765_132000/RConn1 -- T_103088765_132000_/LConn1 -- _CN_103088765_132000_CN_120133940_132000/LConn1
  _CN_111859753_132000_CN_103088765_132000/RConn2 -- T_103088765_132000_/LConn2 -- _CN_103088765_132000_CN_120133940_132000/LConn2
  _CN_111859753_132000_CN_103088765_132000/RConn3 -- T_103088765_132000_/LConn3 -- _CN_103088765_132000_CN_120133940_132000/LConn3 -- bus63/LConn1
  Moen_Lysebotn_kraftstasjon_CN_285928490_132000_CN_296077440_132000/LConn1 -- T_285928490_132000_/LConn1 -- Lyse_2_CN_285928490_132000_CN_50192634_132000/LConn1 -- Lysebotn_Dalen_CN_285928490_132000_CN_289829880_132000/LConn1
  Moen_Lysebotn_kraftstasjon_CN_285928490_132000_CN_296077440_132000/LConn2 -- T_285928490_132000_/LConn2 -- Lyse_2_CN_285928490_132000_CN_50192634_132000/LConn2 -- Lysebotn_Dalen_CN_285928490_132000_CN_289829880_132000/LConn2
  Moen_Lysebotn_kraftstasjon_CN_285928490_132000_CN_296077440_132000/LConn3 -- T_285928490_132000_/LConn3 -- Lyse_2_CN_285928490_132000_CN_50192634_132000/LConn3 -- Lysebotn_Dalen_CN_285928490_132000_CN_289829880_132000/LConn3 -- bus64/LConn1
  Moen_Lysebotn_kraftstasjon_CN_285928490_132000_CN_296077440_132000/RConn1 -- T_296077440_300000_Moen_transformatorstasjon/RConn1 -- L_296077440/LConn1
  Moen_Lysebotn_kraftstasjon_CN_285928490_132000_CN_296077440_132000/RConn2 -- T_296077440_300000_Moen_transformatorstasjon/RConn2 -- L_296077440/LConn2
  Moen_Lysebotn_kraftstasjon_CN_285928490_132000_CN_296077440_132000/RConn3 -- T_296077440_300000_Moen_transformatorstasjon/RConn3 -- L_296077440/LConn3 -- bus65/LConn1
  Lyse_2_CN_285928490_132000_CN_50192634_132000/RConn1 -- T_50192634__Tronsholen/LConn1 -- _CN_50192634_132000_CN_289829886_132000/LConn1 -- _CN_50192634_132000_CN_90273576_132000/LConn1
  Lyse_2_CN_285928490_132000_CN_50192634_132000/RConn2 -- T_50192634__Tronsholen/LConn2 -- _CN_50192634_132000_CN_289829886_132000/LConn2 -- _CN_50192634_132000_CN_90273576_132000/LConn2
  Lyse_2_CN_285928490_132000_CN_50192634_132000/RConn3 -- T_50192634__Tronsholen/LConn3 -- _CN_50192634_132000_CN_289829886_132000/LConn3 -- _CN_50192634_132000_CN_90273576_132000/LConn3 -- bus66/LConn1
  Lysebotn_Dalen_CN_285928490_132000_CN_289829880_132000/RConn1 -- T_289829880__/LConn1 -- Dalen_Forsand_CN_289829880_132000_CN_289829886_132000/LConn1
  Lysebotn_Dalen_CN_285928490_132000_CN_289829880_132000/RConn2 -- T_289829880__/LConn2 -- Dalen_Forsand_CN_289829880_132000_CN_289829886_132000/LConn2
  Lysebotn_Dalen_CN_285928490_132000_CN_289829880_132000/RConn3 -- T_289829880__/LConn3 -- Dalen_Forsand_CN_289829880_132000_CN_289829886_132000/LConn3 -- bus67/LConn1
  Noreledningen_CN_109810733_132000_CN_331597523_132000/LConn1 -- T_109810733_300000;132000_Smestad_trafostasjon/RConn1 -- L_109810733/LConn1
  Noreledningen_CN_109810733_132000_CN_331597523_132000/LConn2 -- T_109810733_300000;132000_Smestad_trafostasjon/RConn2 -- L_109810733/LConn2
  Noreledningen_CN_109810733_132000_CN_331597523_132000/LConn3 -- T_109810733_300000;132000_Smestad_trafostasjon/RConn3 -- L_109810733/LConn3 -- bus68/LConn1
  Noreledningen_CN_109810733_132000_CN_331597523_132000/RConn1 -- T_331597523_132000_/LConn1 -- _CN_331597523_132000_CN_119823786_132000/LConn1
  Noreledningen_CN_109810733_132000_CN_331597523_132000/RConn2 -- T_331597523_132000_/LConn2 -- _CN_331597523_132000_CN_119823786_132000/LConn2
  Noreledningen_CN_109810733_132000_CN_331597523_132000/RConn3 -- T_331597523_132000_/LConn3 -- _CN_331597523_132000_CN_119823786_132000/LConn3 -- bus69/LConn1
  _CN_51854396_132000_CN_122193608_132000/LConn1 -- T_51854396_420000;300000;132000_Tveiten/RConn4 -- L_51854396/LConn1
  _CN_51854396_132000_CN_122193608_132000/LConn2 -- T_51854396_420000;300000;132000_Tveiten/RConn5 -- L_51854396/LConn2
  _CN_51854396_132000_CN_122193608_132000/LConn3 -- T_51854396_420000;300000;132000_Tveiten/RConn6 -- L_51854396/LConn3 -- bus70/LConn1
  _CN_51854396_132000_CN_122193608_132000/RConn1 -- T_122193608_132000_/LConn1 -- _CN_122234000_132000_CN_122193608_132000/LConn1 -- _CN_122193608_132000_CN_107475267_132000/LConn1 -- _CN_122193608_132000_CN_106966310_132000/LConn1
  _CN_51854396_132000_CN_122193608_132000/RConn2 -- T_122193608_132000_/LConn2 -- _CN_122234000_132000_CN_122193608_132000/LConn2 -- _CN_122193608_132000_CN_107475267_132000/LConn2 -- _CN_122193608_132000_CN_106966310_132000/LConn2
  _CN_51854396_132000_CN_122193608_132000/RConn3 -- T_122193608_132000_/LConn3 -- _CN_122234000_132000_CN_122193608_132000/LConn3 -- _CN_122193608_132000_CN_107475267_132000/LConn3 -- _CN_122193608_132000_CN_106966310_132000/LConn3 -- bus71/LConn1
  T_122112073__/LConn1 -- _CN_122112073_132000_CN_325550726_132000/LConn1
  T_122112073__/LConn2 -- _CN_122112073_132000_CN_325550726_132000/LConn2
  _CN_122112073_132000_CN_325550726_132000/LConn3 -- T_122112073__/LConn3 -- bus72/LConn1
  _CN_122112073_132000_CN_325550726_132000/RConn1 -- T_325550726_132000_/LConn1 -- _CN_325550726_132000_CN_291263123_132000/LConn1
  _CN_122112073_132000_CN_325550726_132000/RConn2 -- T_325550726_132000_/LConn2 -- _CN_325550726_132000_CN_291263123_132000/LConn2
  _CN_122112073_132000_CN_325550726_132000/RConn3 -- T_325550726_132000_/LConn3 -- _CN_325550726_132000_CN_291263123_132000/LConn3 -- bus73/LConn1
  _CN_205115991_132000_CN_119823774_132000/LConn1 -- T_205115991_420000;132000_Ringerike_trafostasjon/RConn1 -- _CN_205115991_132000_CN_119823786_132000/LConn1 -- L_205115991/LConn1
  _CN_205115991_132000_CN_119823774_132000/LConn2 -- T_205115991_420000;132000_Ringerike_trafostasjon/RConn2 -- _CN_205115991_132000_CN_119823786_132000/LConn2 -- L_205115991/LConn2
  _CN_205115991_132000_CN_119823774_132000/LConn3 -- T_205115991_420000;132000_Ringerike_trafostasjon/RConn3 -- _CN_205115991_132000_CN_119823786_132000/LConn3 -- L_205115991/LConn3 -- bus74/LConn1
  _CN_205115991_132000_CN_119823774_132000/RConn1 -- T_119823774_132000_/LConn1 -- _CN_330825503_132000_CN_119823774_132000/LConn1
  _CN_205115991_132000_CN_119823774_132000/RConn2 -- T_119823774_132000_/LConn2 -- _CN_330825503_132000_CN_119823774_132000/LConn2
  _CN_205115991_132000_CN_119823774_132000/RConn3 -- T_119823774_132000_/LConn3 -- _CN_330825503_132000_CN_119823774_132000/LConn3 -- bus75/LConn1
  _CN_205115991_132000_CN_119823786_132000/RConn1 -- T_119823786_132000_/LConn1 -- _CN_331597523_132000_CN_119823786_132000/RConn1
  _CN_205115991_132000_CN_119823786_132000/RConn2 -- T_119823786_132000_/LConn2 -- _CN_331597523_132000_CN_119823786_132000/RConn2
  _CN_205115991_132000_CN_119823786_132000/RConn3 -- T_119823786_132000_/LConn3 -- _CN_331597523_132000_CN_119823786_132000/RConn3 -- bus76/LConn1
  T_291263083_132000_Tjøme_transformatorstasjon/LConn1 -- _CN_291263083_132000_CN_291263123_132000/LConn1
  T_291263083_132000_Tjøme_transformatorstasjon/LConn2 -- _CN_291263083_132000_CN_291263123_132000/LConn2
  _CN_291263083_132000_CN_291263123_132000/LConn3 -- T_291263083_132000_Tjøme_transformatorstasjon/LConn3 -- bus77/LConn1
  _CN_291263083_132000_CN_291263123_132000/RConn1 -- T_291263123_132000_/LConn1 -- _CN_325550726_132000_CN_291263123_132000/RConn1 -- _CN_291263123_132000_CN_122228398_132000/LConn1
  _CN_291263083_132000_CN_291263123_132000/RConn2 -- T_291263123_132000_/LConn2 -- _CN_325550726_132000_CN_291263123_132000/RConn2 -- _CN_291263123_132000_CN_122228398_132000/LConn2
  _CN_291263083_132000_CN_291263123_132000/RConn3 -- T_291263123_132000_/LConn3 -- _CN_325550726_132000_CN_291263123_132000/RConn3 -- _CN_291263123_132000_CN_122228398_132000/LConn3 -- bus78/LConn1
  _CN_259135596_132000_CN_432917474_132000/LConn1 -- T_259135596__/RConn1 -- L_259135596/LConn1
  _CN_259135596_132000_CN_432917474_132000/LConn2 -- T_259135596__/RConn2 -- L_259135596/LConn2
  _CN_259135596_132000_CN_432917474_132000/LConn3 -- T_259135596__/RConn3 -- L_259135596/LConn3 -- bus79/LConn1
  _CN_259135596_132000_CN_432917474_132000/RConn1 -- T_432917474__/LConn1 -- _CN_401860888_132000_CN_432917474_132000/LConn1
  _CN_259135596_132000_CN_432917474_132000/RConn2 -- T_432917474__/LConn2 -- _CN_401860888_132000_CN_432917474_132000/LConn2
  _CN_259135596_132000_CN_432917474_132000/RConn3 -- T_432917474__/LConn3 -- _CN_401860888_132000_CN_432917474_132000/LConn3 -- bus80/LConn1
  _CN_329807471_132000_CN_329807474_132000/LConn1 -- T_329807471__/LConn1 -- _CN_329807471_132000_CN_35602245_132000/LConn1
  _CN_329807471_132000_CN_329807474_132000/LConn2 -- T_329807471__/LConn2 -- _CN_329807471_132000_CN_35602245_132000/LConn2
  _CN_329807471_132000_CN_329807474_132000/LConn3 -- T_329807471__/LConn3 -- _CN_329807471_132000_CN_35602245_132000/LConn3 -- bus81/LConn1
  _CN_329807471_132000_CN_329807474_132000/RConn1 -- T_329807474__/LConn1 -- _CN_329807474_132000_CN_329807473_132000/LConn1
  _CN_329807471_132000_CN_329807474_132000/RConn2 -- T_329807474__/LConn2 -- _CN_329807474_132000_CN_329807473_132000/LConn2
  _CN_329807471_132000_CN_329807474_132000/RConn3 -- T_329807474__/LConn3 -- _CN_329807474_132000_CN_329807473_132000/LConn3 -- bus82/LConn1
  _CN_329807471_132000_CN_35602245_132000/RConn1 -- T_35602245_132000_/LConn1 -- _CN_35602245_132000_CN_296269262_132000/LConn1 -- _CN_35602245_132000_CN_296272860_132000/LConn1
  _CN_329807471_132000_CN_35602245_132000/RConn2 -- T_35602245_132000_/LConn2 -- _CN_35602245_132000_CN_296269262_132000/LConn2 -- _CN_35602245_132000_CN_296272860_132000/LConn2
  _CN_329807471_132000_CN_35602245_132000/RConn3 -- T_35602245_132000_/LConn3 -- _CN_35602245_132000_CN_296269262_132000/LConn3 -- _CN_35602245_132000_CN_296272860_132000/LConn3 -- bus83/LConn1
  T_100661361__/LConn1 -- _CN_100661361_132000_CN_100661366_132000/LConn1
  T_100661361__/LConn2 -- _CN_100661361_132000_CN_100661366_132000/LConn2
  _CN_100661361_132000_CN_100661366_132000/LConn3 -- T_100661361__/LConn3 -- bus84/LConn1
  _CN_100661361_132000_CN_100661366_132000/RConn1 -- T_100661366_132000_Hauen_transformatorstasjon/LConn1 -- _CN_100661366_132000_CN_100666299_132000/LConn1 -- _CN_100661366_132000_CN_100655440_132000/LConn1 -- _CN_100661366_132000_CN_325545118_132000/LConn1
  _CN_100661361_132000_CN_100661366_132000/RConn2 -- T_100661366_132000_Hauen_transformatorstasjon/LConn2 -- _CN_100661366_132000_CN_100666299_132000/LConn2 -- _CN_100661366_132000_CN_100655440_132000/LConn2 -- _CN_100661366_132000_CN_325545118_132000/LConn2
  _CN_100661361_132000_CN_100661366_132000/RConn3 -- T_100661366_132000_Hauen_transformatorstasjon/LConn3 -- _CN_100661366_132000_CN_100666299_132000/LConn3 -- bus85/LConn1 -- _CN_100661366_132000_CN_100655440_132000/LConn3 -- _CN_100661366_132000_CN_325545118_132000/LConn3
  _CN_329807474_132000_CN_329807473_132000/RConn1 -- T_329807473__/LConn1 -- _CN_329807476_132000_CN_329807473_132000/LConn1
  _CN_329807474_132000_CN_329807473_132000/RConn2 -- T_329807473__/LConn2 -- _CN_329807476_132000_CN_329807473_132000/LConn2
  _CN_329807474_132000_CN_329807473_132000/RConn3 -- T_329807473__/LConn3 -- _CN_329807476_132000_CN_329807473_132000/LConn3 -- bus86/LConn1
  T_329807476__/LConn1 -- _CN_329807476_132000_CN_329807473_132000/RConn1
  T_329807476__/LConn2 -- _CN_329807476_132000_CN_329807473_132000/RConn2
  _CN_329807476_132000_CN_329807473_132000/RConn3 -- T_329807476__/LConn3 -- bus87/LConn1
  _CN_100661366_132000_CN_100655440_132000/RConn1 -- T_100655440_132000_Meen_koblingsstasjon/LConn1 -- _CN_106966310_132000_CN_100655440_132000/LConn1 -- _CN_100655440_132000_CN_100657505_132000/LConn1
  _CN_100661366_132000_CN_100655440_132000/RConn2 -- T_100655440_132000_Meen_koblingsstasjon/LConn2 -- _CN_106966310_132000_CN_100655440_132000/LConn2 -- _CN_100655440_132000_CN_100657505_132000/LConn2
  _CN_100661366_132000_CN_100655440_132000/RConn3 -- T_100655440_132000_Meen_koblingsstasjon/LConn3 -- _CN_106966310_132000_CN_100655440_132000/LConn3 -- _CN_100655440_132000_CN_100657505_132000/LConn3 -- bus88/LConn1
  _CN_100661366_132000_CN_325545118_132000/RConn1 -- T_325545118_132000_/LConn1 -- _CN_325545118_132000_CN_108634906_132000/LConn1 -- _CN_325545118_132000_CN_435669206_132000/LConn1 -- _CN_325545118_132000_CN_126354422_132000/LConn1 -- _CN_325545118_132000_CN_206538656_132000/LConn1 -- _CN_325545118_132000_CN_100648759_132000/LConn1
  _CN_100661366_132000_CN_325545118_132000/RConn2 -- T_325545118_132000_/LConn2 -- _CN_325545118_132000_CN_108634906_132000/LConn2 -- _CN_325545118_132000_CN_435669206_132000/LConn2 -- _CN_325545118_132000_CN_126354422_132000/LConn2 -- _CN_325545118_132000_CN_206538656_132000/LConn2 -- _CN_325545118_132000_CN_100648759_132000/LConn2
  _CN_100661366_132000_CN_325545118_132000/RConn3 -- T_325545118_132000_/LConn3 -- _CN_325545118_132000_CN_108634906_132000/LConn3 -- _CN_325545118_132000_CN_435669206_132000/LConn3 -- _CN_325545118_132000_CN_126354422_132000/LConn3 -- _CN_325545118_132000_CN_206538656_132000/LConn3 -- _CN_325545118_132000_CN_100648759_132000/LConn3 -- bus89/LConn1
  _CN_100661366_132000_CN_100666299_132000/RConn1 -- T_100666299_132000_/LConn1 -- _CN_325545116_132000_CN_100666299_132000/LConn1 -- _CN_100666299_132000_CN_100666317_132000/LConn1
  _CN_100661366_132000_CN_100666299_132000/RConn2 -- T_100666299_132000_/LConn2 -- _CN_325545116_132000_CN_100666299_132000/LConn2 -- _CN_100666299_132000_CN_100666317_132000/LConn2
  _CN_100661366_132000_CN_100666299_132000/RConn3 -- T_100666299_132000_/LConn3 -- _CN_325545116_132000_CN_100666299_132000/LConn3 -- _CN_100666299_132000_CN_100666317_132000/LConn3 -- bus90/LConn1
  _CN_329807480_132000_CN_296272860_132000/LConn1 -- T_329807480_132000_/LConn1 -- _CN_329807480_132000_CN_329807483_132000/LConn1
  _CN_329807480_132000_CN_296272860_132000/LConn2 -- T_329807480_132000_/LConn2 -- _CN_329807480_132000_CN_329807483_132000/LConn2
  _CN_329807480_132000_CN_296272860_132000/LConn3 -- T_329807480_132000_/LConn3 -- _CN_329807480_132000_CN_329807483_132000/LConn3 -- bus91/LConn1
  _CN_329807480_132000_CN_296272860_132000/RConn1 -- T_296272860_132000_/LConn1 -- _CN_35602245_132000_CN_296272860_132000/RConn1
  _CN_329807480_132000_CN_296272860_132000/RConn2 -- T_296272860_132000_/LConn2 -- _CN_35602245_132000_CN_296272860_132000/RConn2
  _CN_329807480_132000_CN_296272860_132000/RConn3 -- T_296272860_132000_/LConn3 -- _CN_35602245_132000_CN_296272860_132000/RConn3 -- bus92/LConn1
  T_329807483_132000_/LConn1 -- _CN_329807480_132000_CN_329807483_132000/RConn1
  T_329807483_132000_/LConn2 -- _CN_329807480_132000_CN_329807483_132000/RConn2
  _CN_329807480_132000_CN_329807483_132000/RConn3 -- T_329807483_132000_/LConn3 -- bus93/LConn1
  T_120133940__/LConn1 -- _CN_103088765_132000_CN_120133940_132000/RConn1
  T_120133940__/LConn2 -- _CN_103088765_132000_CN_120133940_132000/RConn2
  _CN_103088765_132000_CN_120133940_132000/RConn3 -- T_120133940__/LConn3 -- bus94/LConn1
  _CN_329581505_132000_CN_329581506_132000/LConn1 -- T_329581505_132000_/LConn1 -- _CN_329581505_132000_CN_329581503_132000/LConn1
  _CN_329581505_132000_CN_329581506_132000/LConn2 -- T_329581505_132000_/LConn2 -- _CN_329581505_132000_CN_329581503_132000/LConn2
  _CN_329581505_132000_CN_329581506_132000/LConn3 -- T_329581505_132000_/LConn3 -- _CN_329581505_132000_CN_329581503_132000/LConn3 -- bus95/LConn1
  _CN_329581505_132000_CN_329581506_132000/RConn1 -- T_329581506_132000_/LConn1 -- _CN_329581504_132000_CN_329581506_132000/LConn1
  _CN_329581505_132000_CN_329581506_132000/RConn2 -- T_329581506_132000_/LConn2 -- _CN_329581504_132000_CN_329581506_132000/LConn2
  _CN_329581505_132000_CN_329581506_132000/RConn3 -- T_329581506_132000_/LConn3 -- _CN_329581504_132000_CN_329581506_132000/LConn3 -- bus96/LConn1
  T_329581503_132000_/LConn1 -- _CN_329581505_132000_CN_329581503_132000/RConn1
  T_329581503_132000_/LConn2 -- _CN_329581505_132000_CN_329581503_132000/RConn2
  _CN_329581505_132000_CN_329581503_132000/RConn3 -- T_329581503_132000_/LConn3 -- bus97/LConn1
  _CN_122234000_132000_CN_122234005_132000/LConn1 -- T_122234000_132000_/LConn1 -- _CN_122234000_132000_CN_122229801_132000/LConn1 -- _CN_122234000_132000_CN_122193608_132000/RConn1
  _CN_122234000_132000_CN_122234005_132000/LConn2 -- T_122234000_132000_/LConn2 -- _CN_122234000_132000_CN_122229801_132000/LConn2 -- _CN_122234000_132000_CN_122193608_132000/RConn2
  _CN_122234000_132000_CN_122234005_132000/LConn3 -- T_122234000_132000_/LConn3 -- _CN_122234000_132000_CN_122229801_132000/LConn3 -- _CN_122234000_132000_CN_122193608_132000/RConn3 -- bus98/LConn1
  T_122234005_132000_/LConn1 -- _CN_122234000_132000_CN_122234005_132000/RConn1
  T_122234005_132000_/LConn2 -- _CN_122234000_132000_CN_122234005_132000/RConn2
  _CN_122234000_132000_CN_122234005_132000/RConn3 -- T_122234005_132000_/LConn3 -- bus99/LConn1
  T_122229801_132000_/LConn1 -- _CN_122234000_132000_CN_122229801_132000/RConn1
  T_122229801_132000_/LConn2 -- _CN_122234000_132000_CN_122229801_132000/RConn2
  _CN_122234000_132000_CN_122229801_132000/RConn3 -- T_122229801_132000_/LConn3 -- bus100/LConn1
  T_122228398_132000_/LConn1 -- _CN_291263123_132000_CN_122228398_132000/RConn1
  T_122228398_132000_/LConn2 -- _CN_291263123_132000_CN_122228398_132000/RConn2
  _CN_291263123_132000_CN_122228398_132000/RConn3 -- T_122228398_132000_/LConn3 -- bus101/LConn1
  T_325545116_132000_/LConn1 -- _CN_325545116_132000_CN_100666299_132000/RConn1
  T_325545116_132000_/LConn2 -- _CN_325545116_132000_CN_100666299_132000/RConn2
  _CN_325545116_132000_CN_100666299_132000/RConn3 -- T_325545116_132000_/LConn3 -- bus102/LConn1
  T_108634906__/LConn1 -- _CN_325545118_132000_CN_108634906_132000/RConn1
  T_108634906__/LConn2 -- _CN_325545118_132000_CN_108634906_132000/RConn2
  _CN_325545118_132000_CN_108634906_132000/RConn3 -- T_108634906__/LConn3 -- bus103/LConn1
  T_435669206__/LConn1 -- _CN_325545118_132000_CN_435669206_132000/RConn1
  T_435669206__/LConn2 -- _CN_325545118_132000_CN_435669206_132000/RConn2
  _CN_325545118_132000_CN_435669206_132000/RConn3 -- T_435669206__/LConn3 -- bus104/LConn1
  T_126354422_132000_/LConn1 -- _CN_325545118_132000_CN_126354422_132000/RConn1
  T_126354422_132000_/LConn2 -- _CN_325545118_132000_CN_126354422_132000/RConn2
  _CN_325545118_132000_CN_126354422_132000/RConn3 -- T_126354422_132000_/LConn3 -- bus105/LConn1
  _CN_325545118_132000_CN_206538656_132000/RConn1 -- T_206538656_420000;300000;132000_Rød_transformatorstasjon/RConn4 -- _CN_100677463_132000_CN_206538656_132000/LConn1 -- L_206538656/LConn1
  _CN_325545118_132000_CN_206538656_132000/RConn2 -- T_206538656_420000;300000;132000_Rød_transformatorstasjon/RConn5 -- _CN_100677463_132000_CN_206538656_132000/LConn2 -- L_206538656/LConn2
  _CN_325545118_132000_CN_206538656_132000/RConn3 -- T_206538656_420000;300000;132000_Rød_transformatorstasjon/RConn6 -- _CN_100677463_132000_CN_206538656_132000/LConn3 -- L_206538656/LConn3 -- bus106/LConn1
  _CN_325545118_132000_CN_100648759_132000/RConn1 -- T_100648759_132000_/LConn1 -- _CN_100648754_132000_CN_100648759_132000/LConn1
  _CN_325545118_132000_CN_100648759_132000/RConn2 -- T_100648759_132000_/LConn2 -- _CN_100648754_132000_CN_100648759_132000/LConn2
  _CN_325545118_132000_CN_100648759_132000/RConn3 -- T_100648759_132000_/LConn3 -- _CN_100648754_132000_CN_100648759_132000/LConn3 -- bus107/LConn1
  _CN_128985759_132000_CN_287115460_132000/LConn1 -- T_128985759__/LConn1 -- _CN_128985759_132000_CN_48306065_132000/LConn1
  _CN_128985759_132000_CN_287115460_132000/LConn2 -- T_128985759__/LConn2 -- _CN_128985759_132000_CN_48306065_132000/LConn2
  _CN_128985759_132000_CN_287115460_132000/LConn3 -- T_128985759__/LConn3 -- _CN_128985759_132000_CN_48306065_132000/LConn3 -- bus108/LConn1
  _CN_128985759_132000_CN_287115460_132000/RConn1 -- T_287115460__/RConn1 -- L_287115460/LConn1
  _CN_128985759_132000_CN_287115460_132000/RConn2 -- T_287115460__/RConn2 -- L_287115460/LConn2
  _CN_128985759_132000_CN_287115460_132000/RConn3 -- T_287115460__/RConn3 -- L_287115460/LConn3 -- bus109/LConn1
  _CN_128985759_132000_CN_48306065_132000/RConn1 -- T_48306065__/LConn1 -- _CN_48306065_132000_CN_48310010_132000/LConn1
  _CN_128985759_132000_CN_48306065_132000/RConn2 -- T_48306065__/LConn2 -- _CN_48306065_132000_CN_48310010_132000/LConn2
  _CN_128985759_132000_CN_48306065_132000/RConn3 -- T_48306065__/LConn3 -- _CN_48306065_132000_CN_48310010_132000/LConn3 -- bus110/LConn1
  _CN_355844786_132000_CN_50881349_132000/LConn1 -- T_355844786_300000_Hof_transformator/RConn1 -- L_355844786/LConn1
  _CN_355844786_132000_CN_50881349_132000/LConn2 -- T_355844786_300000_Hof_transformator/RConn2 -- L_355844786/LConn2
  _CN_355844786_132000_CN_50881349_132000/LConn3 -- T_355844786_300000_Hof_transformator/RConn3 -- L_355844786/LConn3 -- bus111/LConn1
  _CN_355844786_132000_CN_50881349_132000/RConn1 -- T_50881349__/LConn1 -- _CN_29322460_132000_CN_50881349_132000/LConn1
  _CN_355844786_132000_CN_50881349_132000/RConn2 -- T_50881349__/LConn2 -- _CN_29322460_132000_CN_50881349_132000/LConn2
  _CN_355844786_132000_CN_50881349_132000/RConn3 -- T_50881349__/LConn3 -- _CN_29322460_132000_CN_50881349_132000/LConn3 -- bus112/LConn1
  T_46832312__/LConn1 -- _CN_46832312_132000_CN_48310010_132000/LConn1
  T_46832312__/LConn2 -- _CN_46832312_132000_CN_48310010_132000/LConn2
  _CN_46832312_132000_CN_48310010_132000/LConn3 -- T_46832312__/LConn3 -- bus113/LConn1
  _CN_46832312_132000_CN_48310010_132000/RConn1 -- T_48310010__/LConn1 -- _CN_48306065_132000_CN_48310010_132000/RConn1
  _CN_46832312_132000_CN_48310010_132000/RConn2 -- T_48310010__/LConn2 -- _CN_48306065_132000_CN_48310010_132000/RConn2
  _CN_46832312_132000_CN_48310010_132000/RConn3 -- T_48310010__/LConn3 -- _CN_48306065_132000_CN_48310010_132000/RConn3 -- bus114/LConn1
  T_107475267_132000_/LConn1 -- _CN_122193608_132000_CN_107475267_132000/RConn1
  T_107475267_132000_/LConn2 -- _CN_122193608_132000_CN_107475267_132000/RConn2
  _CN_122193608_132000_CN_107475267_132000/RConn3 -- T_107475267_132000_/LConn3 -- bus115/LConn1
  _CN_122193608_132000_CN_106966310_132000/RConn1 -- T_106966310_132000_/LConn1 -- _CN_106966310_132000_CN_100655440_132000/RConn1 -- _CN_106966308_132000_CN_106966310_132000/LConn1
  _CN_122193608_132000_CN_106966310_132000/RConn2 -- T_106966310_132000_/LConn2 -- _CN_106966310_132000_CN_100655440_132000/RConn2 -- _CN_106966308_132000_CN_106966310_132000/LConn2
  _CN_122193608_132000_CN_106966310_132000/RConn3 -- T_106966310_132000_/LConn3 -- _CN_106966310_132000_CN_100655440_132000/RConn3 -- bus116/LConn1 -- _CN_106966308_132000_CN_106966310_132000/LConn3
  T_106966308_132000_/LConn1 -- _CN_106966308_132000_CN_106966310_132000/RConn1
  T_106966308_132000_/LConn2 -- _CN_106966308_132000_CN_106966310_132000/RConn2
  _CN_106966308_132000_CN_106966310_132000/RConn3 -- T_106966308_132000_/LConn3 -- bus117/LConn1
  T_29322460_132000_/LConn1 -- _CN_29322460_132000_CN_50881349_132000/RConn1
  T_29322460_132000_/LConn2 -- _CN_29322460_132000_CN_50881349_132000/RConn2
  _CN_29322460_132000_CN_50881349_132000/RConn3 -- T_29322460_132000_/LConn3 -- bus118/LConn1
  _CN_50192634_132000_CN_289829886_132000/RConn1 -- T_289829886__/LConn1 -- Dalen_Forsand_CN_289829880_132000_CN_289829886_132000/RConn1
  _CN_50192634_132000_CN_289829886_132000/RConn2 -- T_289829886__/LConn2 -- Dalen_Forsand_CN_289829880_132000_CN_289829886_132000/RConn2
  _CN_50192634_132000_CN_289829886_132000/RConn3 -- T_289829886__/LConn3 -- Dalen_Forsand_CN_289829880_132000_CN_289829886_132000/RConn3 -- bus119/LConn1
  T_90273576_132000_/LConn1 -- _CN_50192634_132000_CN_90273576_132000/RConn1
  T_90273576_132000_/LConn2 -- _CN_50192634_132000_CN_90273576_132000/RConn2
  _CN_50192634_132000_CN_90273576_132000/RConn3 -- T_90273576_132000_/LConn3 -- bus120/LConn1
  T_90076941_132000_/LConn1 -- _CN_90076941_132000_CN_114336709_132000/LConn1
  T_90076941_132000_/LConn2 -- _CN_90076941_132000_CN_114336709_132000/LConn2
  _CN_90076941_132000_CN_114336709_132000/LConn3 -- T_90076941_132000_/LConn3 -- bus121/LConn1
  _CN_90076941_132000_CN_114336709_132000/RConn1 -- T_114336709_300000;132000_Vang_trafostasjon/RConn1 -- _CN_329581504_132000_CN_114336709_132000/LConn1
  _CN_90076941_132000_CN_114336709_132000/RConn2 -- T_114336709_300000;132000_Vang_trafostasjon/RConn2 -- _CN_329581504_132000_CN_114336709_132000/LConn2
  _CN_90076941_132000_CN_114336709_132000/RConn3 -- T_114336709_300000;132000_Vang_trafostasjon/RConn3 -- _CN_329581504_132000_CN_114336709_132000/LConn3 -- bus122/LConn1
  T_100651279__/LConn1 -- _CN_100651279_132000_CN_100648754_132000/LConn1
  T_100651279__/LConn2 -- _CN_100651279_132000_CN_100648754_132000/LConn2
  _CN_100651279_132000_CN_100648754_132000/LConn3 -- T_100651279__/LConn3 -- bus123/LConn1
  _CN_100651279_132000_CN_100648754_132000/RConn1 -- T_100648754_300000;132000_/RConn1 -- _CN_100648754_132000_CN_100648759_132000/RConn1 -- _CN_100648754_132000_CN_100657505_132000/LConn1 -- L_100648754/LConn1
  _CN_100651279_132000_CN_100648754_132000/RConn2 -- T_100648754_300000;132000_/RConn2 -- _CN_100648754_132000_CN_100648759_132000/RConn2 -- _CN_100648754_132000_CN_100657505_132000/LConn2 -- L_100648754/LConn2
  _CN_100651279_132000_CN_100648754_132000/RConn3 -- T_100648754_300000;132000_/RConn3 -- _CN_100648754_132000_CN_100648759_132000/RConn3 -- _CN_100648754_132000_CN_100657505_132000/LConn3 -- L_100648754/LConn3 -- bus124/LConn1
  _CN_401860888_132000_CN_333991713_132000/RConn1 -- T_401860888_132000_/LConn1 -- _CN_401860888_132000_CN_432917474_132000/RConn1
  _CN_401860888_132000_CN_333991713_132000/RConn2 -- T_401860888_132000_/LConn2 -- _CN_401860888_132000_CN_432917474_132000/RConn2
  _CN_401860888_132000_CN_333991713_132000/RConn3 -- T_401860888_132000_/LConn3 -- _CN_401860888_132000_CN_432917474_132000/RConn3 -- bus125/LConn1
  _CN_330825503_132000_CN_119823774_132000/RConn1 -- T_330825503_300000;132000_/RConn1 -- L_330825503/LConn1
  _CN_330825503_132000_CN_119823774_132000/RConn2 -- T_330825503_300000;132000_/RConn2 -- L_330825503/LConn2
  _CN_330825503_132000_CN_119823774_132000/RConn3 -- T_330825503_300000;132000_/RConn3 -- L_330825503/LConn3 -- bus126/LConn1
  _CN_100648754_132000_CN_100657505_132000/RConn1 -- T_100657505_132000_/LConn1 -- _CN_100655440_132000_CN_100657505_132000/RConn1
  _CN_100648754_132000_CN_100657505_132000/RConn2 -- T_100657505_132000_/LConn2 -- _CN_100655440_132000_CN_100657505_132000/RConn2
  _CN_100648754_132000_CN_100657505_132000/RConn3 -- T_100657505_132000_/LConn3 -- _CN_100655440_132000_CN_100657505_132000/RConn3 -- bus127/LConn1
  _CN_100677463_132000_CN_206538656_132000/RConn1 -- T_100677463_132000_/LConn1 -- _CN_100677463_132000_CN_100666317_132000/LConn1
  _CN_100677463_132000_CN_206538656_132000/RConn2 -- T_100677463_132000_/LConn2 -- _CN_100677463_132000_CN_100666317_132000/LConn2
  _CN_100677463_132000_CN_206538656_132000/RConn3 -- T_100677463_132000_/LConn3 -- _CN_100677463_132000_CN_100666317_132000/LConn3 -- bus128/LConn1
  _CN_100677463_132000_CN_100666317_132000/RConn1 -- T_100666317_132000_/LConn1 -- _CN_100666299_132000_CN_100666317_132000/RConn1
  _CN_100677463_132000_CN_100666317_132000/RConn2 -- T_100666317_132000_/LConn2 -- _CN_100666299_132000_CN_100666317_132000/RConn2
  _CN_100677463_132000_CN_100666317_132000/RConn3 -- T_100666317_132000_/LConn3 -- _CN_100666299_132000_CN_100666317_132000/RConn3 -- bus129/LConn1
  T_296269262__/LConn1 -- _CN_35602245_132000_CN_296269262_132000/RConn1
  T_296269262__/LConn2 -- _CN_35602245_132000_CN_296269262_132000/RConn2
  _CN_35602245_132000_CN_296269262_132000/RConn3 -- T_296269262__/LConn3 -- bus130/LConn1
  _CN_329581504_132000_CN_114336709_132000/RConn1 -- T_329581504_132000_/LConn1 -- _CN_329581504_132000_CN_329581506_132000/RConn1
  _CN_329581504_132000_CN_114336709_132000/RConn2 -- T_329581504_132000_/LConn2 -- _CN_329581504_132000_CN_329581506_132000/RConn2
  _CN_329581504_132000_CN_114336709_132000/RConn3 -- T_329581504_132000_/LConn3 -- _CN_329581504_132000_CN_329581506_132000/RConn3 -- bus131/LConn1
  _CN_296076235_132000_CN_284868564_132000/LConn1 -- T_296076235_300000;132000_/RConn1 -- L_296076235/LConn1
  _CN_296076235_132000_CN_284868564_132000/LConn2 -- T_296076235_300000;132000_/RConn2 -- L_296076235/LConn2
  _CN_296076235_132000_CN_284868564_132000/LConn3 -- T_296076235_300000;132000_/RConn3 -- L_296076235/LConn3 -- bus132/LConn1
  T_284868564_132000_Øye_sekundærstasjon/LConn1 -- _CN_296076235_132000_CN_284868564_132000/RConn1
  T_284868564_132000_Øye_sekundærstasjon/LConn2 -- _CN_296076235_132000_CN_284868564_132000/RConn2
  _CN_296076235_132000_CN_284868564_132000/RConn3 -- T_284868564_132000_Øye_sekundærstasjon/LConn3 -- bus133/LConn1
  Moen_Tonstad_CN_296077440_300000_CN_285825051_300000/LConn1 -- T_296077440_300000_Moen_transformatorstasjon/LConn1 -- Lyse_Duge_CN_296077440_300000_CN_261717967_300000/LConn1 -- Lyse_Førre_CN_296077440_300000_CN_285915728_300000/LConn1
  Moen_Tonstad_CN_296077440_300000_CN_285825051_300000/LConn2 -- T_296077440_300000_Moen_transformatorstasjon/LConn2 -- Lyse_Duge_CN_296077440_300000_CN_261717967_300000/LConn2 -- Lyse_Førre_CN_296077440_300000_CN_285915728_300000/LConn2
  Moen_Tonstad_CN_296077440_300000_CN_285825051_300000/LConn3 -- T_296077440_300000_Moen_transformatorstasjon/LConn3 -- Lyse_Duge_CN_296077440_300000_CN_261717967_300000/LConn3 -- bus134/LConn1 -- Lyse_Førre_CN_296077440_300000_CN_285915728_300000/LConn3
  Moen_Tonstad_CN_296077440_300000_CN_285825051_300000/RConn1 -- T_285825051__/LConn1 -- Tonstad_Stokkeland_CN_285825051_300000_CN_88147266_300000/LConn1 -- Solhom_Tonstad_CN_285825051_300000_CN_295295263_300000/LConn1 -- Tonstad_Feda_CN_285825051_300000_CN_174418125_300000/LConn1
  Moen_Tonstad_CN_296077440_300000_CN_285825051_300000/RConn2 -- T_285825051__/LConn2 -- Tonstad_Stokkeland_CN_285825051_300000_CN_88147266_300000/LConn2 -- Solhom_Tonstad_CN_285825051_300000_CN_295295263_300000/LConn2 -- Tonstad_Feda_CN_285825051_300000_CN_174418125_300000/LConn2
  Moen_Tonstad_CN_296077440_300000_CN_285825051_300000/RConn3 -- T_285825051__/LConn3 -- Tonstad_Stokkeland_CN_285825051_300000_CN_88147266_300000/LConn3 -- bus135/LConn1 -- Solhom_Tonstad_CN_285825051_300000_CN_295295263_300000/LConn3 -- Tonstad_Feda_CN_285825051_300000_CN_174418125_300000/LConn3
  Lyse_Førre_CN_296077440_300000_CN_285915728_300000/RConn1 -- T_285915728__/LConn1 -- Førre_Saurdal_CN_285935887_300000_CN_285915728_300000/LConn1 -- Førre_Hylen_CN_285915728_300000_CN_289304147_300000/LConn1
  Lyse_Førre_CN_296077440_300000_CN_285915728_300000/RConn2 -- T_285915728__/LConn2 -- Førre_Saurdal_CN_285935887_300000_CN_285915728_300000/LConn2 -- Førre_Hylen_CN_285915728_300000_CN_289304147_300000/LConn2
  Lyse_Førre_CN_296077440_300000_CN_285915728_300000/RConn3 -- T_285915728__/LConn3 -- Førre_Saurdal_CN_285935887_300000_CN_285915728_300000/LConn3 -- Førre_Hylen_CN_285915728_300000_CN_289304147_300000/LConn3 -- bus136/LConn1
  Lyse_Duge_CN_296077440_300000_CN_261717967_300000/RConn1 -- T_261717967__/LConn1 -- Roskrepp_Duge_CN_261717967_300000_CN_71356608_300000/LConn1
  Lyse_Duge_CN_296077440_300000_CN_261717967_300000/RConn2 -- T_261717967__/LConn2 -- Roskrepp_Duge_CN_261717967_300000_CN_71356608_300000/LConn2
  Lyse_Duge_CN_296077440_300000_CN_261717967_300000/RConn3 -- T_261717967__/LConn3 -- Roskrepp_Duge_CN_261717967_300000_CN_71356608_300000/LConn3 -- bus137/LConn1
  T_128406208__Sylling_trafostasjon/LConn1 -- Sylling_Hamang_CN_128406208_300000_CN_43078154_300000/LConn1
  T_128406208__Sylling_trafostasjon/LConn2 -- Sylling_Hamang_CN_128406208_300000_CN_43078154_300000/LConn2
  Sylling_Hamang_CN_128406208_300000_CN_43078154_300000/LConn3 -- T_128406208__Sylling_trafostasjon/LConn3 -- bus138/LConn1
  Sylling_Hamang_CN_128406208_300000_CN_43078154_300000/RConn1 -- T_43078154_300000_Hamang_transformatorstasjon/LConn1 -- _CN_43078154_300000_CN_46873771_300000/LConn1
  Sylling_Hamang_CN_128406208_300000_CN_43078154_300000/RConn2 -- T_43078154_300000_Hamang_transformatorstasjon/LConn2 -- _CN_43078154_300000_CN_46873771_300000/LConn2
  Sylling_Hamang_CN_128406208_300000_CN_43078154_300000/RConn3 -- T_43078154_300000_Hamang_transformatorstasjon/LConn3 -- _CN_43078154_300000_CN_46873771_300000/LConn3 -- bus139/LConn1
  _CN_295444099_300000_CN_48798062_300000/LConn1 -- T_295444099_420000;300000;66000_Frogner_transformatorstasjon/RConn1 -- Frogner_Minne_CN_295444099_300000_CN_120279477_300000/LConn1 -- _CN_295444099_300000_CN_113442999_300000/LConn1 -- _CN_295444099_300000_CN_80179519_300000/LConn1
  _CN_295444099_300000_CN_48798062_300000/LConn2 -- T_295444099_420000;300000;66000_Frogner_transformatorstasjon/RConn2 -- Frogner_Minne_CN_295444099_300000_CN_120279477_300000/LConn2 -- _CN_295444099_300000_CN_113442999_300000/LConn2 -- _CN_295444099_300000_CN_80179519_300000/LConn2
  _CN_295444099_300000_CN_48798062_300000/LConn3 -- T_295444099_420000;300000;66000_Frogner_transformatorstasjon/RConn3 -- Frogner_Minne_CN_295444099_300000_CN_120279477_300000/LConn3 -- _CN_295444099_300000_CN_113442999_300000/LConn3 -- _CN_295444099_300000_CN_80179519_300000/LConn3 -- bus140/LConn1
  _CN_295444099_300000_CN_48798062_300000/RConn1 -- T_48798062_300000_Røykås_trafostasjon/LConn1 -- _CN_113442999_300000_CN_48798062_300000/LConn1 -- _CN_114414014_300000_CN_48798062_300000/LConn1
  _CN_295444099_300000_CN_48798062_300000/RConn2 -- T_48798062_300000_Røykås_trafostasjon/LConn2 -- _CN_113442999_300000_CN_48798062_300000/LConn2 -- _CN_114414014_300000_CN_48798062_300000/LConn2
  _CN_295444099_300000_CN_48798062_300000/RConn3 -- T_48798062_300000_Røykås_trafostasjon/LConn3 -- _CN_113442999_300000_CN_48798062_300000/LConn3 -- _CN_114414014_300000_CN_48798062_300000/LConn3 -- bus141/LConn1
  Frogner_Minne_CN_295444099_300000_CN_120279477_300000/RConn1 -- T_120279477_300000;66000_Minne_transformatorstasjon/LConn1 -- Minne_Brenneriroa_CN_120279477_300000_CN_114336709_300000/LConn1
  Frogner_Minne_CN_295444099_300000_CN_120279477_300000/RConn2 -- T_120279477_300000;66000_Minne_transformatorstasjon/LConn2 -- Minne_Brenneriroa_CN_120279477_300000_CN_114336709_300000/LConn2
  Frogner_Minne_CN_295444099_300000_CN_120279477_300000/RConn3 -- T_120279477_300000;66000_Minne_transformatorstasjon/LConn3 -- Minne_Brenneriroa_CN_120279477_300000_CN_114336709_300000/LConn3 -- bus142/LConn1
  _CN_295444099_300000_CN_113442999_300000/RConn1 -- T_113442999_300000_Ulven_trafostasjon/LConn1 -- _CN_113442999_300000_CN_48798062_300000/RConn1
  _CN_295444099_300000_CN_113442999_300000/RConn2 -- T_113442999_300000_Ulven_trafostasjon/LConn2 -- _CN_113442999_300000_CN_48798062_300000/RConn2
  _CN_295444099_300000_CN_113442999_300000/RConn3 -- T_113442999_300000_Ulven_trafostasjon/LConn3 -- _CN_113442999_300000_CN_48798062_300000/RConn3 -- bus143/LConn1
  T_80179519_300000_/LConn1 -- _CN_295444099_300000_CN_80179519_300000/RConn1
  T_80179519_300000_/LConn2 -- _CN_295444099_300000_CN_80179519_300000/RConn2
  _CN_295444099_300000_CN_80179519_300000/RConn3 -- T_80179519_300000_/LConn3 -- bus144/LConn1
  Sauda_Matersdalen_CN_432965765_300000_CN_285805418_300000/LConn1 -- T_432965765__Blåfalli/LConn1 -- _CN_432965765_300000_CN_296078637_300000/LConn1
  Sauda_Matersdalen_CN_432965765_300000_CN_285805418_300000/LConn2 -- T_432965765__Blåfalli/LConn2 -- _CN_432965765_300000_CN_296078637_300000/LConn2
  Sauda_Matersdalen_CN_432965765_300000_CN_285805418_300000/LConn3 -- T_432965765__Blåfalli/LConn3 -- _CN_432965765_300000_CN_296078637_300000/LConn3 -- bus145/LConn1
  Sauda_Matersdalen_CN_432965765_300000_CN_285805418_300000/RConn1 -- T_285805418_300000_/LConn1 -- Sauda_Hylen_CN_289304147_300000_CN_285805418_300000/LConn1 -- _CN_289304185_300000_CN_285805418_300000/LConn1
  Sauda_Matersdalen_CN_432965765_300000_CN_285805418_300000/RConn2 -- T_285805418_300000_/LConn2 -- Sauda_Hylen_CN_289304147_300000_CN_285805418_300000/LConn2 -- _CN_289304185_300000_CN_285805418_300000/LConn2
  Sauda_Matersdalen_CN_432965765_300000_CN_285805418_300000/RConn3 -- T_285805418_300000_/LConn3 -- Sauda_Hylen_CN_289304147_300000_CN_285805418_300000/LConn3 -- _CN_289304185_300000_CN_285805418_300000/LConn3 -- bus146/LConn1
  T_296078637__/LConn1 -- _CN_432965765_300000_CN_296078637_300000/RConn1
  T_296078637__/LConn2 -- _CN_432965765_300000_CN_296078637_300000/RConn2
  _CN_432965765_300000_CN_296078637_300000/RConn3 -- T_296078637__/LConn3 -- bus147/LConn1
  _CN_114845318_300000_CN_114414014_300000/LConn1 -- T_114845318__/LConn1 -- _CN_114845318_300000_CN_290562151_300000/LConn1
  _CN_114845318_300000_CN_114414014_300000/LConn2 -- T_114845318__/LConn2 -- _CN_114845318_300000_CN_290562151_300000/LConn2
  _CN_114845318_300000_CN_114414014_300000/LConn3 -- T_114845318__/LConn3 -- _CN_114845318_300000_CN_290562151_300000/LConn3 -- bus148/LConn1
  _CN_114845318_300000_CN_114414014_300000/RConn1 -- T_114414014_300000_/LConn1 -- _CN_114414014_300000_CN_48798062_300000/RConn1
  _CN_114845318_300000_CN_114414014_300000/RConn2 -- T_114414014_300000_/LConn2 -- _CN_114414014_300000_CN_48798062_300000/RConn2
  _CN_114845318_300000_CN_114414014_300000/RConn3 -- T_114414014_300000_/LConn3 -- _CN_114414014_300000_CN_48798062_300000/RConn3 -- bus149/LConn1
  T_290562151__/LConn1 -- _CN_114845318_300000_CN_290562151_300000/RConn1
  T_290562151__/LConn2 -- _CN_114845318_300000_CN_290562151_300000/RConn2
  _CN_114845318_300000_CN_290562151_300000/RConn3 -- T_290562151__/LConn3 -- bus150/LConn1
  Berheim_Stølaheia_1_CN_166227080_300000_CN_33793216_300000/LConn1 -- T_166227080__/LConn1 -- Stokkeland_Berheim_1_CN_166227080_300000_CN_88147266_300000/LConn1
  Berheim_Stølaheia_1_CN_166227080_300000_CN_33793216_300000/LConn2 -- T_166227080__/LConn2 -- Stokkeland_Berheim_1_CN_166227080_300000_CN_88147266_300000/LConn2
  Berheim_Stølaheia_1_CN_166227080_300000_CN_33793216_300000/LConn3 -- T_166227080__/LConn3 -- Stokkeland_Berheim_1_CN_166227080_300000_CN_88147266_300000/LConn3 -- bus151/LConn1
  T_33793216__Stølaheia_transformatorstasjon/LConn1 -- Berheim_Stølaheia_1_CN_166227080_300000_CN_33793216_300000/RConn1
  T_33793216__Stølaheia_transformatorstasjon/LConn2 -- Berheim_Stølaheia_1_CN_166227080_300000_CN_33793216_300000/RConn2
  Berheim_Stølaheia_1_CN_166227080_300000_CN_33793216_300000/RConn3 -- T_33793216__Stølaheia_transformatorstasjon/LConn3 -- bus152/LConn1
  Stokkeland_Berheim_1_CN_166227080_300000_CN_88147266_300000/RConn1 -- T_88147266_300000;50000_Stokkeland_trafostasjon/LConn1 -- Tonstad_Stokkeland_CN_285825051_300000_CN_88147266_300000/RConn1 -- Kjelland_Stokkeland_CN_124861857_300000_CN_88147266_300000/LConn1
  Stokkeland_Berheim_1_CN_166227080_300000_CN_88147266_300000/RConn2 -- T_88147266_300000;50000_Stokkeland_trafostasjon/LConn2 -- Tonstad_Stokkeland_CN_285825051_300000_CN_88147266_300000/RConn2 -- Kjelland_Stokkeland_CN_124861857_300000_CN_88147266_300000/LConn2
  Stokkeland_Berheim_1_CN_166227080_300000_CN_88147266_300000/RConn3 -- T_88147266_300000;50000_Stokkeland_trafostasjon/LConn3 -- Tonstad_Stokkeland_CN_285825051_300000_CN_88147266_300000/RConn3 -- Kjelland_Stokkeland_CN_124861857_300000_CN_88147266_300000/LConn3 -- bus153/LConn1
  _CN_43078154_300000_CN_46873771_300000/RConn1 -- T_46873771_300000_Bærum_trafostasjon/LConn1 -- _CN_46873771_300000_CN_109810733_300000/LConn1
  _CN_43078154_300000_CN_46873771_300000/RConn2 -- T_46873771_300000_Bærum_trafostasjon/LConn2 -- _CN_46873771_300000_CN_109810733_300000/LConn2
  _CN_43078154_300000_CN_46873771_300000/RConn3 -- T_46873771_300000_Bærum_trafostasjon/LConn3 -- _CN_46873771_300000_CN_109810733_300000/LConn3 -- bus154/LConn1
  _CN_287115458_300000_CN_288685602_300000/LConn1 -- T_287115458__/LConn1 -- _CN_287115458_300000_CN_355844786_300000/LConn1 -- _CN_287115458_300000_CN_287115460_300000/LConn1
  _CN_287115458_300000_CN_288685602_300000/LConn2 -- T_287115458__/LConn2 -- _CN_287115458_300000_CN_355844786_300000/LConn2 -- _CN_287115458_300000_CN_287115460_300000/LConn2
  _CN_287115458_300000_CN_288685602_300000/LConn3 -- T_287115458__/LConn3 -- _CN_287115458_300000_CN_355844786_300000/LConn3 -- bus155/LConn1 -- _CN_287115458_300000_CN_287115460_300000/LConn3
  _CN_287115458_300000_CN_288685602_300000/RConn1 -- T_288685602__/LConn1 -- Rjukan_Songa_CN_288685602_300000_CN_288812256_300000/LConn1
  _CN_287115458_300000_CN_288685602_300000/RConn2 -- T_288685602__/LConn2 -- Rjukan_Songa_CN_288685602_300000_CN_288812256_300000/LConn2
  _CN_287115458_300000_CN_288685602_300000/RConn3 -- T_288685602__/LConn3 -- Rjukan_Songa_CN_288685602_300000_CN_288812256_300000/LConn3 -- bus156/LConn1
  T_287115460__/LConn1 -- _CN_287115458_300000_CN_287115460_300000/RConn1
  T_287115460__/LConn2 -- _CN_287115458_300000_CN_287115460_300000/RConn2
